simulink library "AEMS_Standard_Library"  (R2016b)
settings: Solver=ode45  StartTime=0.0  StopTime=10.0  RelTol=1e-3
undefined symbols (not defined in the file or in its folder): BkPY, carto, Cbx_extegr, Cbx_lpegrsys, Cbx_portegr, Cnx_bnk_nr_conf, Cnx_cyl_nr_conf, ConfigManagement, configuration_management, Cxx_dcm_io_tmr_end_xxxx, Cxx_dcm_rt_tmr_end, Cxx_DID_xxxx_IO_max, Cxx_DID_xxxx_IO_min, Cxx_egrhsofs, Cxx_vmaniegi, DEM_DEBOUNCE_FREEZE, DEM_DTR_CTL_INVISIBLE, DEM_DTR_CTL_NORMAL, Dem_DtrId2_XXX, Dem_DtrId3_XXX, Dem_DtrId4_XXX, Dem_DtrId5_XXX, Dem_DtrId6_XXX, Dem_DtrId7_XXX, Dem_DtrId8_XXX, Dem_DtrId9_XXX, Dem_DtrId_XXX, Dem_EnableConditionId2_XXX, Dem_EnableConditionId3_XXX, Dem_EnableConditionId4_XXX, Dem_EnableConditionId5_XXX, Dem_EnableConditionId6_XXX, Dem_EnableConditionId7_XXX, Dem_EnableConditionId8_XXX, Dem_EnableConditionId_XXX, Dem_EventId, Dem_EventId2_XXX, Dem_EventId3_XXX, Dem_EventId4_XXX, Dem_EventId5_XXX, Dem_EventId6_XXX, Dem_EventId7_XXX, Dem_EventId8_XXX, Dem_EventId9_XXX, Dem_EventId_Device_Faulttype, Dem_EventId_XXX, DEM_IUMPR_GENERAL_DENOMINATOR, DEM_OPCYC_IGNITION, Dem_RatioId2_XXX, Dem_RatioId3_XXX, Dem_RatioId4_XXX, Dem_RatioId5_XXX, Dem_RatioId6_XXX, Dem_RatioId7_XXX, Dem_RatioId8_XXX, Dem_RatioId_XXX, Dem_StorageConditionId2_XXX, Dem_StorageConditionId3_XXX, Dem_StorageConditionId4_XXX, Dem_StorageConditionId5_XXX ... (+65)
libraries: AEMS_Standard_Library x477, simulink x2
(part 10 of 39)

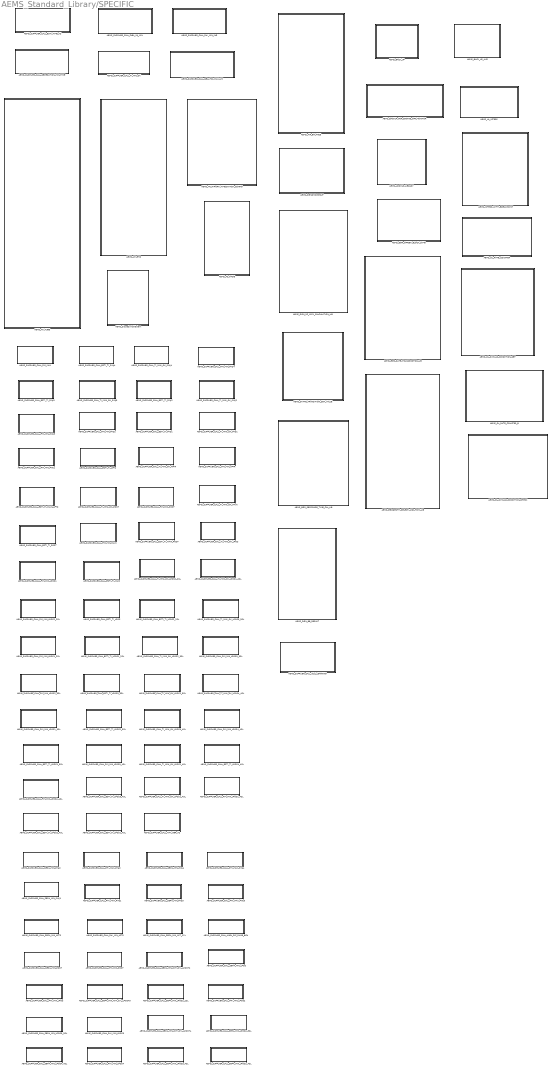
== system AEMS_Standard_Library/SPECIFIC ==
  AEMS_AIR_BALANCE : Subsystem  Tag=[LIB]  Description=User library of air balance calculation  mask(AEMS_AIR_BALANCE){Cnx_cyl_nr_conf=Cnx_cyl_nr_conf, Cbx_portegr=Cbx_portegr, Cbx_extegr=Cbx_extegr, Cxx_vmaniegi=Cxx_vmaniegi, Cbx_lpegrsys=Cbx_lpegrsys}
      mask prompts: Cnx_cyl_nr_conf "iCYLNDER"; Cbx_portegr "mfPORTEGR"; Cbx_extegr "mfEXTEGR"; Cxx_vmaniegi "mVMANIEGI"; Cbx_lpegrsys "mfLPEGRSYS"
      mask help:
      | Air Balance Block.
      | Use only at 2ms.
      settings: AttributesFormatString=%<MaskType>
      mask Help:
      | eval('path_lib=fileparts(which(''AEMS_Standard_Library''));');
      | doc_path = [path_lib '\help\AEMS_AIR_BALANCE.pdf'];
      | eval('open(doc_path)')
      mask Display: disp('AEMS_AIR_BALANCE')
  AEMS_AS_PADE : Subsystem  Tag=[LIB]  Description=|  TreatAsAtomicUnit=on  RTWFcnName=RSA_AS_Pade  mask(AEMS_AS_PADE){Cxb_lb_dly_t_para=Cxb_lb_dly_t_para, Cxp_lb_b0_1=Cxp_lb_b0_1, Cxp_lb_b1_1=Cxp_lb_b1_1, Cxp_lb_a1_1=Cxp_lb_a1_1, Cxp_lb_a2_1=Cxp_lb_a2_1, Cxp_lb_b0_2=Cxp_lb_b0_2, Cxp_lb_b1_2=Cxp_lb_b1_2, Cxp_lb_a1_2=Cxp_lb_a1_2, Cxp_lb_a2_2=Cxp_lb_a2_2, Cxp_lb_b0_3=Cxp_lb_b0_3, Cxp_lb_b1_3=Cxp_lb_b1_3, Cxp_lb_a1_3=Cxp_lb_a1_3, Cxp_lb_a2_3=Cxp_lb_a2_3}
      | This bloc describes a 6th-order Pade approximation of time delays.  It can be used to model dead times or transport delays in many processes.
      |                                                                                                                                              
      |  Inputs:                                                                                                                                     
      | Vbx_dly_ena:	 Boolean that enables the Pade delay model                                                                                      
      | Vbx_dly_init_ena:Boolean that initiates the Pade delay model                                                                                 
      | Vxx_dly_t:	delay time to be applied on the input signal (s)                                                                                  
      | Vxx_ftc_frst_order:	constant time of the upstream first order filter of Pade approximation  (s)                                              
      | Vxx_in:	 input signal to be delayed (kg/h)                                                                                                   
      |                                                                                                                                              
      | Outputs:                                                                                                                                     
      | Vxx_in_dly:            the approximation of delay time on the filtered input signal (kg/h)                                                   
      | Vxx_in_fil:              the input signal filtered by the first order filter (kg/h)
      mask help:
      | This block describes a 6th-order Pade approximation of time delays.  It can be used to model dead times or transport delays in many processes.
      |
      | Inputs:
      | Vbx_dly_init_ena:                Boolean that initiates the Pade delay model
      | Vxx_dly_t:                       Delay time to be applied on the input signal (s)
      | Vxx_ftc_frst_order:              Constant time of the upstream first order filter of Pade approximation  (s)
      | Vxx_in:                          Input signal to be delayed (kg/h)or (mg/strk)
      | Timestep:                        Time input that initiates the Pade delay model
      |
      | Outputs:
      | Vxx_in_dly:                      The approximation of delay time on the filtered input signal (kg/h) or (mg/strk)
      | Vxx_in_fil:                      The input signal filtered by the first order filter (kg/h) or (mg/strk)
      settings: AttributesFormatString=%<MaskType>\nCxb_lb_dly_t_para = %<Cxb_lb_dly_t_para>\nCxp_lb_b0_1 = %<Cxp_lb_b0_1>\nCxp_lb_b1_1 = %<Cxp_lb_b1_1>\nCxp_lb_a1_1 = %<Cxp_lb_a1_1>\nCxp_lb_a2_1 = %<Cxp_lb_a2_1>\nCxp_lb_b0_2 = %<Cxp_lb_b0_2>\nCxp_lb_b1_2 = %<Cxp_lb_b1_2>\nCxp_lb_a1_2 = %<Cxp_lb_a1_2>\nCxp_lb_a2_2 = %<Cxp_lb_a2_2>\nCxp_lb_b0_3 = %<Cxp_lb_b0_3>\nCxp_lb_b1_3 = %<Cxp_lb_b1_3>\nCxp_lb_a1_3 = %<Cxp_lb_a1_3>\nCxp_lb_a2_3 = %<Cxp_lb_a2_3>  RTWFcnNameOpts=User specified
      mask Help:
      | eval('path_lib=fileparts(which(''AEMS_Standard_Library''));');
      | mskblk=get_param(gcbh,'MaskType');
      | doc_path = [path_lib '\Help\',mskblk,'.pdf'];
      | eval('open(doc_path)');
      mask Display: disp('AEMS_AS_PADE\n\n')
  AEMS_AT_EHR : Subsystem  Tag=[LIB]  RTWFcnName=RSA_AT_ehr  mask(AEMS_AT_EHR){Den_Tol=1.1920929e-07}
      mask prompts: Den_Tol "Denominator Tolerance"
      mask help:
      | Library : thermal model
      | This function computes an energetic balance of the considered system. It estimates the brick temperature, the energy incoming, the energy leaving, the loss by external convection and the energy
      | created in the system.
      |
      | Version : 01.00
      settings: AttributesFormatString=%<MaskType>\nDenominator Tolerance=%<Den_Tol>  RTWFcnNameOpts=User specified
      mask Help:
      | eval('path_lib=fileparts(which(''AEMS_Standard_Library''));');
      | mskblk=get_param(gcbh,'MaskType');
      | doc_path = [path_lib '\Help\',mskblk,'.pdf'];
      | eval('open(doc_path)');
      mask Display: disp('AEMS_AT_EHR')
  AEMS_AT_TUBE : Subsystem  Tag=[LIB]  Description=|  RTWFcnName=RSA_AT_tube  mask(AEMS_AT_TUBE){Den_Tol=1.1920929e-07}
      | This block determines the exhaust gas downstream temperature, the temperature of the tube material,
      | the thermal power lost by the tube material and the thermal power lost by the gas inside the tube.
      mask prompts: Den_Tol "Denominator Tolerance"
      mask help:
      | This block determines the exhaust gas downstream temperature, the temperature of the tube material,
      | the thermal power lost by the tube material and the thermal power lost by the gas inside the tube.
      |
      | Version :01.00
      settings: AttributesFormatString=%<MaskType>\nDenominator Tolerance = %<Den_Tol>  RTWFcnNameOpts=User specified
      mask Help:
      | eval('path_lib=fileparts(which(''AEMS_Standard_Library''));');
      | mskblk=get_param(gcbh,'MaskType');
      | doc_path = [path_lib '\Help\',mskblk,'.pdf'];
      | eval('open(doc_path)');
      mask Display: disp('AEMS_AT_TUBE')
  AEMS_BACKUP_FOR_ENGINE_OFF_MONITOR : Subsystem  Tag=[LIB]  mask(AEMS_BACKUP_FOR_ENGINE_OFF_MONITOR){}
      mask help: This block is for Monitoring the Engine OFF condition.
      settings: AttributesFormatString=%<MaskType>
      mask Help:
      | eval('path_lib=fileparts(which(''AEMS_Standard_Library''));');
      | doc_path = [path_lib '\help\AEMS_BACKUP_FOR_ENGINE_OFF_MONITOR.pdf'];
      | eval('open(doc_path)')
      mask Display: disp('AEMS_BACKUP_FOR_ENGINE_OFF_MONITOR')
  AEMS_BACK_UP : Subsystem  Tag=[LIB]  mask(AEMS_BACK_UP){max_parameter=max, min_parameter=min}
      mask prompts: max_parameter "max"; min_parameter "min"
      mask init:
      | name=get_param(gcb,'MaskValueString');
      | name=sprintf(strrep(name,'|','\n'));
      | name=strread(name,'%s','delimiter',',');
      settings: AttributesFormatString=%<MaskType>\nmax = %<max_parameter>\nmin = %<min_parameter>
      mask Help:
      | eval('path_lib=fileparts(which(''AEMS_Standard_Library''));');
      | doc_path = [path_lib '\help\AEMS_BACK_UP.pdf'];
      | eval('open(doc_path)')
      mask Display: disp('AEMS_BACK_UP')
  AEMS_BACK_UP_AVE : Subsystem  Tag=[LIB]  mask(AEMS_BACK_UP_AVE){max_parameter=max, min_parameter=min}
      mask prompts: max_parameter "max"; min_parameter "min"
      mask init:
      | name=get_param(gcb,'MaskValueString');
      | name=sprintf(strrep(name,'|','\n'));
      | name=strread(name,'%s','delimiter',',');
      settings: AttributesFormatString=%<MaskType>\nmax = %<max_parameter>\nmin = %<min_parameter>
      mask Help:
      | eval('path_lib=fileparts(which(''AEMS_Standard_Library''));');
      | doc_path = [path_lib '\help\AEMS_BACK_UP_AVE.pdf'];
      | eval('open(doc_path)')
      mask Display: disp('AEMS_BACK_UP_AVE')
  AEMS_DGNDMDPGCUT : Subsystem  Tag=[LIB]  mask(AEMS_DGNDMDPGCUT){}
      settings: AttributesFormatString=%<MaskType>
      mask Help:
      | eval('path_lib=fileparts(which(''AEMS_Standard_Library''));');
      | doc_path = [path_lib '\help\AEMS_DGNDMDPGCUT.pdf'];
      | eval('open(doc_path)')
      mask Display: disp('AEMS_DGNDMDPGCUT')
  AEMS_DGN_BB_RESULT : Subsystem  Tag=[LIB]  mask(AEMS_DGN_BB_RESULT){}
      settings: AttributesFormatString=%<MaskType>
      mask Help:
      | eval('path_lib=fileparts(which(''AEMS_Standard_Library''));');
      | doc_path = [path_lib '\help\AEMS_DGN_BB_RESULT.pdf'];
      | eval('open(doc_path)')
      mask Display: disp('AEMS_DGN_BB_RESULT')
  AEMS_DGN_MF_MISX_CALCULATION_LIB : Subsystem  Tag=[LIB]  mask(AEMS_DGN_MF_MISX_CALCULATION_LIB){}
      settings: AttributesFormatString=%<MaskType>
      mask Help:
      | eval('path_lib=fileparts(which(''AEMS_Standard_Library''));');
      | doc_path = [path_lib '\help\AEMS_DGN_MF_MISX_CALCULATION_LIB.pdf'];
      | eval('open(doc_path)')
      mask Display: disp('AEMS_DGN_MF_MISX_CALCULATION_LIB')
  AEMS_EGRQESTH_SELECT_AND_TRIM_LIB : Subsystem  Tag=[LIB]  mask(AEMS_EGRQESTH_SELECT_AND_TRIM_LIB){}
      settings: AttributesFormatString=%<MaskType>
      mask Help:
      | eval('path_lib=fileparts(which(''AEMS_Standard_Library''));');
      | doc_path = [path_lib '\help\AEMS_EGRQESTH_SELECT_AND_TRIM_LIB.pdf'];
      | eval('open(doc_path)')
      mask Display: disp('AEMS_EGRQESTH_SELECT_AND_TRIM_LIB')
  AEMS_EGR_OFFSET_BLOCK_DIM8 : Subsystem  Tag=[LIB]  mask(AEMS_EGR_OFFSET_BLOCK_DIM8){Cxx_egrhsofs=0}
      mask prompts: Cxx_egrhsofs "mEGRHSOFS"
      settings: AttributesFormatString=%<MaskType>
      mask Help:
      | eval('path_lib=fileparts(which(''AEMS_Standard_Library''));');
      | doc_path = [path_lib '\help\AEMS_EGR_OFFSET_BLOCK_DIM8.pdf'];
      | eval('open(doc_path)')
      mask Display: disp('AEMS_EGR_OFFSET_BLOCK_DIM8')
  AEMS_EGR_RATE_TRANSPORTOR_LIB : Subsystem  Tag=[LIB]  Description=This USER LIBRARY calculates EGR rate delay of each part.  mask(AEMS_EGR_RATE_TRANSPORTOR_LIB){}
      mask help: This USER LIBRARY calculates EGR rate delay of each part.
      settings: AttributesFormatString=%<MaskType>
      mask Help:
      | eval('path_lib=fileparts(which(''AEMS_Standard_Library''));');
      | doc_path = [path_lib '\help\AEMS_EGR_RATE_TRANSPORTOR_LIB.pdf'];
      | eval('open(doc_path)')
      mask Display: disp('AEMS_EGR_RATE_TRANSPORTOR_LIB')
  AEMS_EGR_RESPONSE_TIME_CAL_LIB : Subsystem  Tag=[LIB]  mask(AEMS_EGR_RESPONSE_TIME_CAL_LIB){}
      settings: AttributesFormatString=%<MaskType>
      mask Help:
      | eval('path_lib=fileparts(which(''AEMS_Standard_Library''));');
      | doc_path = [path_lib '\help\AEMS_EGR_RESPONSE_TIME_CAL_LIB.pdf'];
      | eval('open(doc_path)')
      mask Display: disp('AEMS_EGR_RESPONSE_TIME_CAL_LIB')
  AEMS_INTERP_WITH_BREAKPOINT : Subsystem  Tag=[LIB]  mask(AEMS_INTERP_WITH_BREAKPOINT){}
      settings: AttributesFormatString=%<MaskType>
      mask Help:
      | eval('path_lib=fileparts(which(''AEMS_Standard_Library''));');
      | doc_path = [path_lib '\help\AEMS_INTERP_WITH_BREAKPOINT.pdf'];
      | eval('open(doc_path)')
      mask Display: disp('AEMS_INTERP_WITH_BREAKPOINT')
  AEMS_LOOKUP_LIBRARY : Subsystem  Tag=[LIB]  mask(AEMS_LOOKUP_LIBRARY){}
      settings: AttributesFormatString=%<MaskType>
      mask Help:
      | eval('path_lib=fileparts(which(''AEMS_Standard_Library''));');
      | doc_path = [path_lib '\help\AEMS_LOOKUP_LIBRARY.pdf'];
      | eval('open(doc_path)')
      mask Display: disp('AEMS_LOOKUP_LIBRARY')
  AEMS_MULTIPORT_TIMESWITCH_CONFIG : Subsystem  Tag=[LIB]  mask(AEMS_MULTIPORT_TIMESWITCH_CONFIG){LimitDimInputs=8}
      mask prompts: LimitDimInputs "Limit of Dimension of Inputs"
      mask help:
      | This switch allows to switch among inputs regrouped in a vector using Selector. It provides a smooth transition between the previously selected input and the currently selected input over a duration.
      | It should be noted that during the transition, the current value of both inputs is taken into account and not just values at the moment of switching.
      |
      | As a result, discontinuities can arise if a new input is seleted before the previous transition has ended.
      |
      | [INPUTS]
      | Duration: Transition duration
      | Select_Input: Select an input in the vector Inputs
      | Inputs: Regrouped inputs
      | dT: Sample time
      |
      | [OUTPUTS]
      | Output: Smooth value from previous and current selected inputs
      | Slop_on: indicate that there is a switch
      |
      | [PARAMETERS]
      | LimitNumberInputs: Limit number of input signals regrouped in Inputs
      settings: AttributesFormatString=|
      | %<MaskType>
      | Limit Dimension of Inputs : %<LimitDimInputs>
      mask Help:
      | eval('path_lib=fileparts(which(''lib_dcmap_sdt''));');
      | doc_path = [path_lib '\help\AEMS_MULTIPORT_TIMESWITCH_CONFIG.pdf'];
      | eval('open(doc_path)')
      mask Display: disp('AEMS_MULTIPORT_TIMESWITCH_CONFIG')
  AEMS_OL_RATE_COUNTER : Subsystem  Tag=[LIB]  mask(AEMS_OL_RATE_COUNTER){}
      settings: AttributesFormatString=%<MaskType>
      mask Help:
      | eval('path_lib=fileparts(which(''AEMS_Standard_Library''));');
      | doc_path = [path_lib '\help\AEMS_OL_RATE_COUNTER.pdf'];
      | eval('open(doc_path)')
      mask Display: disp('AEMS_OL_RATE_COUNTER')
  AEMS_OL_RATE_COUNTER_B : Subsystem  Tag=[LIB]  mask(AEMS_OL_RATE_COUNTER_B){}
      settings: AttributesFormatString=%<MaskType>
      mask Help:
      | eval('path_lib=fileparts(which(''AEMS_Standard_Library''));');
      | doc_path = [path_lib '\help\AEMS_OL_RATE_COUNTER_B.pdf'];
      | eval('open(doc_path)')
      mask Display: disp('AEMS_OL_RATE_COUNTER_B')
  AEMS_OL_SIMILAR_CONDITION_CHECK : Subsystem  Tag=[LIB]  mask(AEMS_OL_SIMILAR_CONDITION_CHECK){}
      settings: AttributesFormatString=%<MaskType>
      mask Help:
      | eval('path_lib=fileparts(which(''AEMS_Standard_Library''));');
      | doc_path = [path_lib '\help\AEMS_OL_SIMILAR_CONDITION_CHECK.pdf'];
      | eval('open(doc_path)')
      mask Display: disp('AEMS_OL_SIMILAR_CONDITION_CHECK')
  AEMS_OL_SIMILAR_CONDITION_SET : Subsystem  Tag=[LIB]  mask(AEMS_OL_SIMILAR_CONDITION_SET){}
      settings: AttributesFormatString=%<MaskType>
      mask Help:
      | eval('path_lib=fileparts(which(''AEMS_Standard_Library''));');
      | doc_path = [path_lib '\help\AEMS_OL_SIMILAR_CONDITION_SET.pdf'];
      | eval('open(doc_path)')
      mask Display: disp('AEMS_OL_SIMILAR_CONDITION_SET')
  AEMS_STATE_TRANSITION_SET_VALUE : Subsystem  Tag=[LIB]  mask(AEMS_STATE_TRANSITION_SET_VALUE){}
      settings: AttributesFormatString=%<MaskType>
      mask Help:
      | eval('path_lib=fileparts(which(''AEMS_Standard_Library''));');
      | doc_path = [path_lib '\help\AEMS_STATE_TRANSITION_SET_VALUE.pdf'];
      | eval('open(doc_path)')
      mask Display: disp('AEMS_STATE_TRANSITION_SET_VALUE')
  AEMS_SUPPLIER_CALL_ANGL_DIF_SAME_BCH : Subsystem  Tag=[LIB]  TreatAsAtomicUnit=on  RTWFcnName=SUPPLIER_CALL_Angl_dif_same_bch  mask(AEMS_SUPPLIER_CALL_ANGL_DIF_SAME_BCH){}
      mask help: Angle without injection command between 2 cylinder ordered by the same bench.
      mask init:
      | Thisblk = gcb;
      | model_type_pos = strsplit(Thisblk,'/');%to split all the layer paths in order to get the runnable path
      | runnable_path = [bdroot '/' model_type_pos{2}];%to get the runnable or AIPCALL path
      | trg_port_name = get_param(find_system(runnable_path,'BlockType','TriggerPort'),'Name');%to get the function call trigger name
      | TaskRate = '';%the raster suffix is stored in the parameter 
      | 
      | if ~isempty(trg_port_name)
      |     trg_port_name_spltd = strsplit(trg_port_name{1},'_');%splitting is done in order to get the raster and its type(Sched or Event)
      |     
      |     % checking for rasters of type Sched or Event especially occuring in
      |     % runnables
      |     if ~isempty(regexp(trg_port_name_spltd{1},'^Sched|^Event','once')) 
      |         TaskRate = ['_' regexprep(trg_port_name_spltd{1},'Sched|Event','','once')];
      |         
      |     %checking if the raster is dcmcb and this is applicable only for
      |     %APICALL
      |     elseif ~isempty(regexp([trg_port_name_spltd{1} '_' trg_port_name_spltd{2} '_' ],'^DataServices_DCM_|^RoutineServices_DCM_','once'))||...
      |             ~isempty(regexp(trg_port_name_spltd{1},'^Dcm$','once'))
      |         TaskRate = '_dcmcb';
      |         
      |     %checking if this block is used under the function call trigger
      |     %starting with "Com" and then giving an error message
      |     %this is applicable only for APICALL
      |     elseif ~isempty(regexp(trg_port_name_spltd{1},'^Com$','once'))
      |         msg = sprintf(['\n','The Supplier call block "' Thisblk '" should not be present within APICALLs having function call trigger as "Com"']);
      |         errordlg(msg);
      |         return;
      |     end
      | end
      | 
      | DataName = ['Supplier_call_angl_dif_nxt_cyl' TaskRate];%the variable name that should be given to DataStoreRead block 
      | set_param([Thisblk '/DataStoreRead'],'DataStoreName',DataName);%Setting the DataStoreName of DataStoreRead block
      | 
      | %other settings done to this variable name
      | structVxx=Simulink.Signal;
      | structVxx.Dimensions=1;
      | structVxx.DimensionsMode='Fixed';
      | structVxx.DataType='single';
      | structVxx.Complexity='real';
      | structVxx.SamplingMode='Sample based';
      | structVxx.SampleTime=-1;
      | assignin('base',DataName,structVxx);
      settings: AttributesFormatString=%<MaskType>  RTWSystemCode=Nonreusable function  RTWFcnNameOpts=User specified
      mask Help:
      | eval('path_lib=fileparts(which(''AEMS_Standard_Library''));');
      | mskblk=get_param(gcbh,'MaskType');
      | doc_path = [path_lib '\Help\',mskblk,'.pdf'];
      | eval('open(doc_path)');
  AEMS_SUPPLIER_CALL_ESTI_TIME_INJ : Subsystem  Tag=[LIB]  TreatAsAtomicUnit=on  RTWFcnName=SUPPLIER_CALL_Esti_ti_main_post3  mask(AEMS_SUPPLIER_CALL_ESTI_TIME_INJ){Outportname=Vxx_fms_esti_ti_wish_main_post2, Suppliercallname=SUPPLIER_CALL_Esti_ti_main_post2, Splitnum=2}
      mask prompts: Outportname "Outport Name"; Suppliercallname "Supplier call Name"; Splitnum "Split"
      mask help:
      | Estimation of time of injection, depending on rail pressure, on fuel quantity and of fuel density.
      |
      | Each block will be translated into code C by this way:
      | Output=Supplier call API Name(In,Splitnum);
      | Example for Supplier_Call_Esti_ti_main_post3, corresponding output variable is Vxx_fms_esti_ti_wish_main_post3
      | Vxx_fms_esti_ti_wish_main_post3= Supplier_Call_Esti_ti_main_post3(In,3);
      mask init:
      | ThisBlk = gcb;
      | OutPorts            =   {'Vxx_fms_esti_ti_post1','Vxx_fms_esti_ti_post1_2sl','Vxx_fms_esti_ti_post1_3sl','Vxx_fms_esti_ti_post2_2sl','Vxx_fms_esti_ti_post2_3sl',...
      |                     'Vxx_fms_esti_ti_post3_3sl','Vxx_fms_esti_ti_wish_main_post1','Vxx_fms_esti_ti_wish_main_post2','Vxx_fms_esti_ti_wish_main_post3'};
      | 
      | Supplier_Calls      =   {'SUPPLIER_CALL_Esti_ti_post1','SUPPLIER_CALL_Esti_ti_post1','SUPPLIER_CALL_Esti_ti_post1','SUPPLIER_CALL_Esti_ti_post2','SUPPLIER_CALL_Esti_ti_post2',...
      |                           'SUPPLIER_CALL_Esti_ti_post3','SUPPLIER_CALL_Esti_ti_main_post1','SUPPLIER_CALL_Esti_ti_main_post2','SUPPLIER_CALL_Esti_ti_main_post3'};
      | 
      | Data_Names         =   {'Supplier_Call_Esti_ti_post1','Supplier_Call_Esti_ti_post1','Supplier_Call_Esti_ti_post1','Supplier_Call_Esti_ti_post2','Supplier_Call_Esti_ti_post2',...
      |                           'Supplier_Call_Esti_ti_post3','Supplier_Call_Esti_ti_main_post1','Supplier_Call_Esti_ti_main_post2','Supplier_Call_Esti_ti_main_post3'};                      
      |                       
      |                       
      | Splits              =   {'1','2','3','2','3','3','1','2','3'};
      | 
      | model_type_pos = strsplit(ThisBlk,'/');
      | runnable_path = [bdroot '/' model_type_pos{2}];%to get the runnable or AIPCALL path
      | trg_port_name = get_param(find_system(runnable_path,'BlockType','TriggerPort'),'Name');%to get the function call trigger name
      | TaskRate = '';
      | if ~isempty(trg_port_name)
      |     trg_port_name_spltd = strsplit(trg_port_name{1},'_');
      |     if ~isempty(regexp(trg_port_name_spltd{1},'^Sched|^Event','once'))
      |         TaskRate = ['_' regexprep(trg_port_name_spltd{1},'Sched|Event','','once')];
      |     elseif ~isempty(regexp([trg_port_name_spltd{1} '_' trg_port_name_spltd{2} '_' ],'^DataServices_DCM_|^RoutineServices_DCM_','once'))||...
      |             ~isempty(regexp(trg_port_name_spltd{1},'^Dcm$','once'))
      |         TaskRate = '_dcmcb';
      |     elseif ~isempty(regexp(trg_port_name_spltd{1},'^Com$','once'))
      |         msg = sprintf(['\n','The Supplier call block "' Thisblk '" should not be present within APICALLs having function call trigger as "Com"']);
      |         errordlg(msg);
      |         return;
      |     end
      | end
      | 
      | Idx_Of_Outportname = find(ismember(OutPorts,Outportname));
      | DataName = [Data_Names{Idx_Of_Outportname} TaskRate];
      | 
      | %set the  suppliername according to the Outport name.
      | set_param(ThisBlk,'Suppliercallname',Supplier_Calls{Idx_Of_Outportname});
      | set_param(ThisBlk,'Splitnum',Splits{Idx_Of_Outportname});
      | 
      | %Get the paths of the blks under this lib block.
      | Const_Blk = [ThisBlk,'/Splitnum'];%%path of "const block" inside this lib blk.
      | DSR_Blk   = [ThisBlk,'/Data_Store_Read'];%path of "Data store read block" inside this lib blk.
      | Outport_Blk = find_system(ThisBlk,'LookUnderMasks','all','FollowLinks','on','BlockType','Outport');
      | Outport_Blk = Outport_Blk{1};%I know this is d only outport blk.
      | 
      | %set the attributes of the blks under this lib block, based on teh Outportname chosen by d user.
      | set_param(Outport_Blk,'Name',Outportname);
      | set_param(DSR_Blk,'DataStoreName',DataName);
      | set_param(Const_Blk,'Value',Splits{Idx_Of_Outportname});
      | 
      | %To create a singal object in d base workspace.
      | EvalStr = ['exist(''',DataName,''',''var'')'];
      | structVxx=Simulink.Signal;
      | structVxx.Dimensions=1;
      | structVxx.DimensionsMode='Fixed';
      | structVxx.DataType='single';
      | structVxx.Complexity='real';
      | structVxx.SamplingMode='Sample based';
      | structVxx.SampleTime=-1;
      | isDefined= evalin('base',EvalStr);%This line checks whether the DataName exist in the base workspace.
      | if (isDefined==0)
      |     assignin('base',DataName,structVxx);
      | end
      settings: RTWSystemCode=Inline  RTWFcnNameOpts=User specified
      settings: AttributesFormatString=|
      | %<MaskType>
      | Supplier Call Name = %<Suppliercallname>
      | Outport Name = %<Outportname>
      | Split Number = %<Splitnum>
      mask Help:
      | eval('path_lib=fileparts(which(''AEMS_Standard_Library''));');
      | mskblk=get_param(gcbh,'MaskType');
      | doc_path = [path_lib '\Help\',mskblk,'.pdf'];
      | eval('open(doc_path)');
      mask TypeOptions Outportname: Vxx_fms_esti_ti_post1 | Vxx_fms_esti_ti_post1_2sl | Vxx_fms_esti_ti_post1_3sl | Vxx_fms_esti_ti_post2_2sl | Vxx_fms_esti_ti_post2_3sl | Vxx_fms_esti_ti_post3_3sl | Vxx_fms_esti_ti_wish_main_post1 | Vxx_fms_esti_ti_wish_main_post2 | Vxx_fms_esti_ti_wish_main_post3
      mask Callback Outportname:
      | OutPorts            =   {'Vxx_fms_esti_ti_post1','Vxx_fms_esti_ti_post1_2sl','Vxx_fms_esti_ti_post1_3sl','Vxx_fms_esti_ti_post2_2sl','Vxx_fms_esti_ti_post2_3sl',...
      |                     'Vxx_fms_esti_ti_post3_3sl','Vxx_fms_esti_ti_wish_main_post1','Vxx_fms_esti_ti_wish_main_post2','Vxx_fms_esti_ti_wish_main_post3'};
      | 
      | Supplier_Calls      =   {'SUPPLIER_CALL_Esti_ti_post1','SUPPLIER_CALL_Esti_ti_post1','SUPPLIER_CALL_Esti_ti_post1','SUPPLIER_CALL_Esti_ti_post2','SUPPLIER_CALL_Esti_ti_post2',...
      |                           'SUPPLIER_CALL_Esti_ti_post3','SUPPLIER_CALL_Esti_ti_main_post1','SUPPLIER_CALL_Esti_ti_main_post2','SUPPLIER_CALL_Esti_ti_main_post3'};
      | 
      | Splits              =   {'1','2','3','2','3','3','1','2','3'};
      | 
      | Outportname = get_param(gcb,'Outportname');
      | 
      | Idx_Of_Outportname = find(ismember(OutPorts,Outportname));
      | %set the  suppliername according to the Outport name.
      | set_param(gcb,'Suppliercallname',Supplier_Calls{Idx_Of_Outportname});
      | set_param(gcb,'Splitnum',Splits{Idx_Of_Outportname});
      | cellfun(@clear,{'Idx_Of_Outportname','Outportname','OutPorts','Splits','Supplier_Calls'});
  AEMS_SUPPLIER_CALL_ESTI_TI_AFTR : Subsystem  Tag=[LIB]  TreatAsAtomicUnit=on  RTWFcnName=SUPPLIER_CALL_Esti_ti_aftr  mask(AEMS_SUPPLIER_CALL_ESTI_TI_AFTR){}
      mask help:
      | Estimation of time of injection, depending on rail pressure, on fuel quantity and of fuel density
      |
      | This block is to call Supplier call API.
      mask init:
      | Thisblk = gcb;
      | model_type_pos = strsplit(Thisblk,'/');%to split all the layer paths in order to get the runnable path
      | runnable_path = [bdroot '/' model_type_pos{2}];%to get the runnable or AIPCALL path
      | trg_port_name = get_param(find_system(runnable_path,'BlockType','TriggerPort'),'Name');%to get the function call trigger name
      | TaskRate = '';%the raster suffix is stored in the parameter 
      | 
      | if ~isempty(trg_port_name)
      |     trg_port_name_spltd = strsplit(trg_port_name{1},'_');%splitting is done in order to get the raster and its type(Sched or Event)
      |     
      |     % checking for rasters of type Sched or Event especially occuring in
      |     % runnables
      |     if ~isempty(regexp(trg_port_name_spltd{1},'^Sched|^Event','once')) 
      |         TaskRate = ['_' regexprep(trg_port_name_spltd{1},'Sched|Event','','once')];
      |         
      |     %checking if the raster is dcmcb and this is applicable only for
      |     %APICALL
      |     elseif ~isempty(regexp([trg_port_name_spltd{1} '_' trg_port_name_spltd{2} '_' ],'^DataServices_DCM_|^RoutineServices_DCM_','once'))||...
      |             ~isempty(regexp(trg_port_name_spltd{1},'^Dcm$','once'))
      |         TaskRate = '_dcmcb';
      |         
      |     %checking if this block is used under the function call trigger
      |     %starting with "Com" and then giving an error message
      |     %this is applicable only for APICALL
      |     elseif ~isempty(regexp(trg_port_name_spltd{1},'^Com$','once'))
      |         msg = sprintf(['\n','The Supplier call block "' Thisblk '" should not be present within APICALLs having function call trigger as "Com"']);
      |         errordlg(msg);
      |         return;
      |     end
      | end
      | 
      | DataName = ['Supplier_call_esti_ti_aftr' TaskRate];%the variable name that should be given to DataStoreRead block 
      | set_param([Thisblk '/DataStoreRead'],'DataStoreName',DataName);%Setting the DataStoreName of DataStoreRead block
      | 
      | %other settings done to this variable name
      | structVxx=Simulink.Signal;
      | structVxx.Dimensions=1;
      | structVxx.DimensionsMode='Fixed';
      | structVxx.DataType='single';
      | structVxx.Complexity='real';
      | structVxx.SamplingMode='Sample based';
      | structVxx.SampleTime=-1;
      | assignin('base',DataName,structVxx);
      settings: AttributesFormatString=%<MaskType>  RTWSystemCode=Nonreusable function  RTWFcnNameOpts=User specified
      mask Help:
      | eval('path_lib=fileparts(which(''AEMS_Standard_Library''));');
      | mskblk=get_param(gcbh,'MaskType');
      | doc_path = [path_lib '\Help\',mskblk,'.pdf'];
      | eval('open(doc_path)');
  AEMS_SUPPLIER_CALL_ESTI_TI_LPOS : Subsystem  Tag=[LIB]  TreatAsAtomicUnit=on  RTWFcnName=SUPPLIER_CALL_Esti_ti_lpos  mask(AEMS_SUPPLIER_CALL_ESTI_TI_LPOS){}
      mask help:
      | Estimation of time of injection, depending on rail pressure, on fuel quantity and of fuel density
      |
      | This block is to call Supplier call API.
      mask init:
      | Thisblk = gcb;
      | model_type_pos = strsplit(Thisblk,'/');%to split all the layer paths in order to get the runnable path
      | runnable_path = [bdroot '/' model_type_pos{2}];%to get the runnable or AIPCALL path
      | trg_port_name = get_param(find_system(runnable_path,'BlockType','TriggerPort'),'Name');%to get the function call trigger name
      | TaskRate = '';%the raster suffix is stored in the parameter 
      | 
      | if ~isempty(trg_port_name)
      |     trg_port_name_spltd = strsplit(trg_port_name{1},'_');%splitting is done in order to get the raster and its type(Sched or Event)
      |     
      |     % checking for rasters of type Sched or Event especially occuring in
      |     % runnables
      |     if ~isempty(regexp(trg_port_name_spltd{1},'^Sched|^Event','once')) 
      |         TaskRate = ['_' regexprep(trg_port_name_spltd{1},'Sched|Event','','once')];
      |         
      |     %checking if the raster is dcmcb and this is applicable only for
      |     %APICALL
      |     elseif ~isempty(regexp([trg_port_name_spltd{1} '_' trg_port_name_spltd{2} '_' ],'^DataServices_DCM_|^RoutineServices_DCM_','once'))||...
      |             ~isempty(regexp(trg_port_name_spltd{1},'^Dcm$','once'))
      |         TaskRate = '_dcmcb';
      |         
      |     %checking if this block is used under the function call trigger
      |     %starting with "Com" and then giving an error message
      |     %this is applicable only for APICALL
      |     elseif ~isempty(regexp(trg_port_name_spltd{1},'^Com$','once'))
      |         msg = sprintf(['\n','The Supplier call block "' Thisblk '" should not be present within APICALLs having function call trigger as "Com"']);
      |         errordlg(msg);
      |         return;
      |     end
      | end
      | 
      | DataName = ['Supplier_call_esti_ti_lpos' TaskRate];%the variable name that should be given to DataStoreRead block 
      | set_param([Thisblk '/DataStoreRead'],'DataStoreName',DataName);%Setting the DataStoreName of DataStoreRead block
      | 
      | %other settings done to this variable name
      | structVxx=Simulink.Signal;
      | structVxx.Dimensions=1;
      | structVxx.DimensionsMode='Fixed';
      | structVxx.DataType='single';
      | structVxx.Complexity='real';
      | structVxx.SamplingMode='Sample based';
      | structVxx.SampleTime=-1;
      | assignin('base',DataName,structVxx);
      settings: AttributesFormatString=%<MaskType>  RTWSystemCode=Nonreusable function  RTWFcnNameOpts=User specified
      mask Help:
      | eval('path_lib=fileparts(which(''AEMS_Standard_Library''));');
      | mskblk=get_param(gcbh,'MaskType');
      | doc_path = [path_lib '\Help\',mskblk,'.pdf'];
      | eval('open(doc_path)');
  AEMS_SUPPLIER_CALL_ESTI_TI_LPOS1_2SL : Subsystem  Tag=[LIB]  TreatAsAtomicUnit=on  RTWFcnName=SUPPLIER_CALL_Esti_ti_lpos1_2sl  mask(AEMS_SUPPLIER_CALL_ESTI_TI_LPOS1_2SL){}
      mask help:
      | Estimation of time of injection, depending on rail pressure, on fuel quantity and of fuel density
      |
      | This block is to call Supplier call API.
      mask init:
      | Thisblk = gcb;
      | model_type_pos = strsplit(Thisblk,'/');%to split all the layer paths in order to get the runnable path
      | runnable_path = [bdroot '/' model_type_pos{2}];%to get the runnable or AIPCALL path
      | trg_port_name = get_param(find_system(runnable_path,'BlockType','TriggerPort'),'Name');%to get the function call trigger name
      | TaskRate = '';%the raster suffix is stored in the parameter 
      | 
      | if ~isempty(trg_port_name)
      |     trg_port_name_spltd = strsplit(trg_port_name{1},'_');%splitting is done in order to get the raster and its type(Sched or Event)
      |     
      |     % checking for rasters of type Sched or Event especially occuring in
      |     % runnables
      |     if ~isempty(regexp(trg_port_name_spltd{1},'^Sched|^Event','once')) 
      |         TaskRate = ['_' regexprep(trg_port_name_spltd{1},'Sched|Event','','once')];
      |         
      |     %checking if the raster is dcmcb and this is applicable only for
      |     %APICALL
      |     elseif ~isempty(regexp([trg_port_name_spltd{1} '_' trg_port_name_spltd{2} '_' ],'^DataServices_DCM_|^RoutineServices_DCM_','once'))||...
      |             ~isempty(regexp(trg_port_name_spltd{1},'^Dcm$','once'))
      |         TaskRate = '_dcmcb';
      |         
      |     %checking if this block is used under the function call trigger
      |     %starting with "Com" and then giving an error message
      |     %this is applicable only for APICALL
      |     elseif ~isempty(regexp(trg_port_name_spltd{1},'^Com$','once'))
      |         msg = sprintf(['\n','The Supplier call block "' Thisblk '" should not be present within APICALLs having function call trigger as "Com"']);
      |         errordlg(msg);
      |         return;
      |     end
      | end
      | 
      | DataName = ['Supplier_call_esti_ti_lpos1_2sl' TaskRate];%the variable name that should be given to DataStoreRead block 
      | set_param([Thisblk '/DataStoreRead'],'DataStoreName',DataName);%Setting the DataStoreName of DataStoreRead block
      | 
      | %other settings done to this variable name
      | structVxx=Simulink.Signal;
      | structVxx.Dimensions=1;
      | structVxx.DimensionsMode='Fixed';
      | structVxx.DataType='single';
      | structVxx.Complexity='real';
      | structVxx.SamplingMode='Sample based';
      | structVxx.SampleTime=-1;
      | assignin('base',DataName,structVxx);
      settings: AttributesFormatString=%<MaskType>  RTWSystemCode=Nonreusable function  RTWFcnNameOpts=User specified
      mask Help:
      | eval('path_lib=fileparts(which(''AEMS_Standard_Library''));');
      | mskblk=get_param(gcbh,'MaskType');
      | doc_path = [path_lib '\Help\',mskblk,'.pdf'];
      | eval('open(doc_path)');
  AEMS_SUPPLIER_CALL_ESTI_TI_LPOS1_3SL : Subsystem  Tag=[LIB]  TreatAsAtomicUnit=on  RTWFcnName=SUPPLIER_CALL_Esti_ti_lpos1_3sl  mask(AEMS_SUPPLIER_CALL_ESTI_TI_LPOS1_3SL){}
      mask help:
      | Estimation of time of injection, depending on rail pressure, on fuel quantity and of fuel density
      |
      | This block is to call Supplier call API.
      mask init:
      | Thisblk = gcb;
      | model_type_pos = strsplit(Thisblk,'/');%to split all the layer paths in order to get the runnable path
      | runnable_path = [bdroot '/' model_type_pos{2}];%to get the runnable or AIPCALL path
      | trg_port_name = get_param(find_system(runnable_path,'BlockType','TriggerPort'),'Name');%to get the function call trigger name
      | TaskRate = '';%the raster suffix is stored in the parameter 
      | 
      | if ~isempty(trg_port_name)
      |     trg_port_name_spltd = strsplit(trg_port_name{1},'_');%splitting is done in order to get the raster and its type(Sched or Event)
      |     
      |     % checking for rasters of type Sched or Event especially occuring in
      |     % runnables
      |     if ~isempty(regexp(trg_port_name_spltd{1},'^Sched|^Event','once')) 
      |         TaskRate = ['_' regexprep(trg_port_name_spltd{1},'Sched|Event','','once')];
      |         
      |     %checking if the raster is dcmcb and this is applicable only for
      |     %APICALL
      |     elseif ~isempty(regexp([trg_port_name_spltd{1} '_' trg_port_name_spltd{2} '_' ],'^DataServices_DCM_|^RoutineServices_DCM_','once'))||...
      |             ~isempty(regexp(trg_port_name_spltd{1},'^Dcm$','once'))
      |         TaskRate = '_dcmcb';
      |         
      |     %checking if this block is used under the function call trigger
      |     %starting with "Com" and then giving an error message
      |     %this is applicable only for APICALL
      |     elseif ~isempty(regexp(trg_port_name_spltd{1},'^Com$','once'))
      |         msg = sprintf(['\n','The Supplier call block "' Thisblk '" should not be present within APICALLs having function call trigger as "Com"']);
      |         errordlg(msg);
      |         return;
      |     end
      | end
      | 
      | DataName = ['Supplier_call_esti_ti_lpos1_3sl' TaskRate];%the variable name that should be given to DataStoreRead block 
      | set_param([Thisblk '/DataStoreRead'],'DataStoreName',DataName);%Setting the DataStoreName of DataStoreRead block
      | 
      | %other settings done to this variable name
      | structVxx=Simulink.Signal;
      | structVxx.Dimensions=1;
      | structVxx.DimensionsMode='Fixed';
      | structVxx.DataType='single';
      | structVxx.Complexity='real';
      | structVxx.SamplingMode='Sample based';
      | structVxx.SampleTime=-1;
      | assignin('base',DataName,structVxx);
      settings: AttributesFormatString=%<MaskType>  RTWSystemCode=Nonreusable function  RTWFcnNameOpts=User specified
      mask Help:
      | eval('path_lib=fileparts(which(''AEMS_Standard_Library''));');
      | mskblk=get_param(gcbh,'MaskType');
      | doc_path = [path_lib '\Help\',mskblk,'.pdf'];
      | eval('open(doc_path)');
  AEMS_SUPPLIER_CALL_ESTI_TI_LPOS1_4SL : Subsystem  Tag=[LIB]  TreatAsAtomicUnit=on  RTWFcnName=SUPPLIER_CALL_Esti_ti_lpos1_4sl  mask(AEMS_SUPPLIER_CALL_ESTI_TI_LPOS1_4SL){}
      mask help:
      | Estimation of time of injection, depending on rail pressure, on fuel quantity and of fuel density
      |
      | This block is to call Supplier call API.
      mask init:
      | Thisblk = gcb;
      | model_type_pos = strsplit(Thisblk,'/');%to split all the layer paths in order to get the runnable path
      | runnable_path = [bdroot '/' model_type_pos{2}];%to get the runnable or AIPCALL path
      | trg_port_name = get_param(find_system(runnable_path,'BlockType','TriggerPort'),'Name');%to get the function call trigger name
      | TaskRate = '';%the raster suffix is stored in the parameter 
      | 
      | if ~isempty(trg_port_name)
      |     trg_port_name_spltd = strsplit(trg_port_name{1},'_');%splitting is done in order to get the raster and its type(Sched or Event)
      |     
      |     % checking for rasters of type Sched or Event especially occuring in
      |     % runnables
      |     if ~isempty(regexp(trg_port_name_spltd{1},'^Sched|^Event','once')) 
      |         TaskRate = ['_' regexprep(trg_port_name_spltd{1},'Sched|Event','','once')];
      |         
      |     %checking if the raster is dcmcb and this is applicable only for
      |     %APICALL
      |     elseif ~isempty(regexp([trg_port_name_spltd{1} '_' trg_port_name_spltd{2} '_' ],'^DataServices_DCM_|^RoutineServices_DCM_','once'))||...
      |             ~isempty(regexp(trg_port_name_spltd{1},'^Dcm$','once'))
      |         TaskRate = '_dcmcb';
      |         
      |     %checking if this block is used under the function call trigger
      |     %starting with "Com" and then giving an error message
      |     %this is applicable only for APICALL
      |     elseif ~isempty(regexp(trg_port_name_spltd{1},'^Com$','once'))
      |         msg = sprintf(['\n','The Supplier call block "' Thisblk '" should not be present within APICALLs having function call trigger as "Com"']);
      |         errordlg(msg);
      |         return;
      |     end
      | end
      | 
      | DataName = ['Supplier_call_esti_ti_lpos1_4sl' TaskRate];%the variable name that should be given to DataStoreRead block 
      | set_param([Thisblk '/DataStoreRead'],'DataStoreName',DataName);%Setting the DataStoreName of DataStoreRead block
      | 
      | %other settings done to this variable name
      | structVxx=Simulink.Signal;
      | structVxx.Dimensions=1;
      | structVxx.DimensionsMode='Fixed';
      | structVxx.DataType='single';
      | structVxx.Complexity='real';
      | structVxx.SamplingMode='Sample based';
      | structVxx.SampleTime=-1;
      | assignin('base',DataName,structVxx);
      settings: AttributesFormatString=%<MaskType>  RTWSystemCode=Nonreusable function  RTWFcnNameOpts=User specified
      mask Help:
      | eval('path_lib=fileparts(which(''AEMS_Standard_Library''));');
      | mskblk=get_param(gcbh,'MaskType');
      | doc_path = [path_lib '\Help\',mskblk,'.pdf'];
      | eval('open(doc_path)');
  AEMS_SUPPLIER_CALL_ESTI_TI_LPOS2_2SL : Subsystem  Tag=[LIB]  TreatAsAtomicUnit=on  RTWFcnName=SUPPLIER_CALL_Esti_ti_lpos2_2sl  mask(AEMS_SUPPLIER_CALL_ESTI_TI_LPOS2_2SL){}
      mask help:
      | Estimation of time of injection, depending on rail pressure, on fuel quantity and of fuel density
      |
      | This block is to call Supplier call API.
      mask init:
      | Thisblk = gcb;
      | model_type_pos = strsplit(Thisblk,'/');%to split all the layer paths in order to get the runnable path
      | runnable_path = [bdroot '/' model_type_pos{2}];%to get the runnable or AIPCALL path
      | trg_port_name = get_param(find_system(runnable_path,'BlockType','TriggerPort'),'Name');%to get the function call trigger name
      | TaskRate = '';%the raster suffix is stored in the parameter 
      | 
      | if ~isempty(trg_port_name)
      |     trg_port_name_spltd = strsplit(trg_port_name{1},'_');%splitting is done in order to get the raster and its type(Sched or Event)
      |     
      |     % checking for rasters of type Sched or Event especially occuring in
      |     % runnables
      |     if ~isempty(regexp(trg_port_name_spltd{1},'^Sched|^Event','once')) 
      |         TaskRate = ['_' regexprep(trg_port_name_spltd{1},'Sched|Event','','once')];
      |         
      |     %checking if the raster is dcmcb and this is applicable only for
      |     %APICALL
      |     elseif ~isempty(regexp([trg_port_name_spltd{1} '_' trg_port_name_spltd{2} '_' ],'^DataServices_DCM_|^RoutineServices_DCM_','once'))||...
      |             ~isempty(regexp(trg_port_name_spltd{1},'^Dcm$','once'))
      |         TaskRate = '_dcmcb';
      |         
      |     %checking if this block is used under the function call trigger
      |     %starting with "Com" and then giving an error message
      |     %this is applicable only for APICALL
      |     elseif ~isempty(regexp(trg_port_name_spltd{1},'^Com$','once'))
      |         msg = sprintf(['\n','The Supplier call block "' Thisblk '" should not be present within APICALLs having function call trigger as "Com"']);
      |         errordlg(msg);
      |         return;
      |     end
      | end
      | 
      | DataName = ['Supplier_call_esti_ti_lpos2_2sl' TaskRate];%the variable name that should be given to DataStoreRead block 
      | set_param([Thisblk '/DataStoreRead'],'DataStoreName',DataName);%Setting the DataStoreName of DataStoreRead block
      | 
      | %other settings done to this variable name
      | structVxx=Simulink.Signal;
      | structVxx.Dimensions=1;
      | structVxx.DimensionsMode='Fixed';
      | structVxx.DataType='single';
      | structVxx.Complexity='real';
      | structVxx.SamplingMode='Sample based';
      | structVxx.SampleTime=-1;
      | assignin('base',DataName,structVxx);
      settings: AttributesFormatString=%<MaskType>  RTWSystemCode=Nonreusable function  RTWFcnNameOpts=User specified
      mask Help:
      | eval('path_lib=fileparts(which(''AEMS_Standard_Library''));');
      | mskblk=get_param(gcbh,'MaskType');
      | doc_path = [path_lib '\Help\',mskblk,'.pdf'];
      | eval('open(doc_path)');
  AEMS_SUPPLIER_CALL_ESTI_TI_LPOS2_3SL : Subsystem  Tag=[LIB]  TreatAsAtomicUnit=on  RTWFcnName=SUPPLIER_CALL_Esti_ti_lpos2_3sl  mask(AEMS_SUPPLIER_CALL_ESTI_TI_LPOS2_3SL){}
      mask help:
      | Estimation of time of injection, depending on rail pressure, on fuel quantity and of fuel density
      |
      | This block is to call Supplier call API.
      mask init:
      | Thisblk = gcb;
      | model_type_pos = strsplit(Thisblk,'/');%to split all the layer paths in order to get the runnable path
      | runnable_path = [bdroot '/' model_type_pos{2}];%to get the runnable or AIPCALL path
      | trg_port_name = get_param(find_system(runnable_path,'BlockType','TriggerPort'),'Name');%to get the function call trigger name
      | TaskRate = '';%the raster suffix is stored in the parameter 
      | 
      | if ~isempty(trg_port_name)
      |     trg_port_name_spltd = strsplit(trg_port_name{1},'_');%splitting is done in order to get the raster and its type(Sched or Event)
      |     
      |     % checking for rasters of type Sched or Event especially occuring in
      |     % runnables
      |     if ~isempty(regexp(trg_port_name_spltd{1},'^Sched|^Event','once')) 
      |         TaskRate = ['_' regexprep(trg_port_name_spltd{1},'Sched|Event','','once')];
      |         
      |     %checking if the raster is dcmcb and this is applicable only for
      |     %APICALL
      |     elseif ~isempty(regexp([trg_port_name_spltd{1} '_' trg_port_name_spltd{2} '_' ],'^DataServices_DCM_|^RoutineServices_DCM_','once'))||...
      |             ~isempty(regexp(trg_port_name_spltd{1},'^Dcm$','once'))
      |         TaskRate = '_dcmcb';
      |         
      |     %checking if this block is used under the function call trigger
      |     %starting with "Com" and then giving an error message
      |     %this is applicable only for APICALL
      |     elseif ~isempty(regexp(trg_port_name_spltd{1},'^Com$','once'))
      |         msg = sprintf(['\n','The Supplier call block "' Thisblk '" should not be present within APICALLs having function call trigger as "Com"']);
      |         errordlg(msg);
      |         return;
      |     end
      | end
      | 
      | DataName = ['Supplier_call_esti_ti_lpos2_3sl' TaskRate];%the variable name that should be given to DataStoreRead block 
      | set_param([Thisblk '/DataStoreRead'],'DataStoreName',DataName);%Setting the DataStoreName of DataStoreRead block
      | 
      | %other settings done to this variable name
      | structVxx=Simulink.Signal;
      | structVxx.Dimensions=1;
      | structVxx.DimensionsMode='Fixed';
      | structVxx.DataType='single';
      | structVxx.Complexity='real';
      | structVxx.SamplingMode='Sample based';
      | structVxx.SampleTime=-1;
      | assignin('base',DataName,structVxx);
      settings: AttributesFormatString=%<MaskType>  RTWSystemCode=Nonreusable function  RTWFcnNameOpts=User specified
      mask Help:
      | eval('path_lib=fileparts(which(''AEMS_Standard_Library''));');
      | mskblk=get_param(gcbh,'MaskType');
      | doc_path = [path_lib '\Help\',mskblk,'.pdf'];
      | eval('open(doc_path)');
  AEMS_SUPPLIER_CALL_ESTI_TI_LPOS2_4SL : Subsystem  Tag=[LIB]  TreatAsAtomicUnit=on  RTWFcnName=SUPPLIER_CALL_Esti_ti_lpos2_4sl  mask(AEMS_SUPPLIER_CALL_ESTI_TI_LPOS2_4SL){}
      mask help:
      | Estimation of time of injection, depending on rail pressure, on fuel quantity and of fuel density
      |
      | This block is to call Supplier call API.
      mask init:
      | Thisblk = gcb;
      | model_type_pos = strsplit(Thisblk,'/');%to split all the layer paths in order to get the runnable path
      | runnable_path = [bdroot '/' model_type_pos{2}];%to get the runnable or AIPCALL path
      | trg_port_name = get_param(find_system(runnable_path,'BlockType','TriggerPort'),'Name');%to get the function call trigger name
      | TaskRate = '';%the raster suffix is stored in the parameter 
      | 
      | if ~isempty(trg_port_name)
      |     trg_port_name_spltd = strsplit(trg_port_name{1},'_');%splitting is done in order to get the raster and its type(Sched or Event)
      |     
      |     % checking for rasters of type Sched or Event especially occuring in
      |     % runnables
      |     if ~isempty(regexp(trg_port_name_spltd{1},'^Sched|^Event','once')) 
      |         TaskRate = ['_' regexprep(trg_port_name_spltd{1},'Sched|Event','','once')];
      |         
      |     %checking if the raster is dcmcb and this is applicable only for
      |     %APICALL
      |     elseif ~isempty(regexp([trg_port_name_spltd{1} '_' trg_port_name_spltd{2} '_' ],'^DataServices_DCM_|^RoutineServices_DCM_','once'))||...
      |             ~isempty(regexp(trg_port_name_spltd{1},'^Dcm$','once'))
      |         TaskRate = '_dcmcb';
      |         
      |     %checking if this block is used under the function call trigger
      |     %starting with "Com" and then giving an error message
      |     %this is applicable only for APICALL
      |     elseif ~isempty(regexp(trg_port_name_spltd{1},'^Com$','once'))
      |         msg = sprintf(['\n','The Supplier call block "' Thisblk '" should not be present within APICALLs having function call trigger as "Com"']);
      |         errordlg(msg);
      |         return;
      |     end
      | end
      | 
      | DataName = ['Supplier_call_esti_ti_lpos2_4sl' TaskRate];%the variable name that should be given to DataStoreRead block 
      | set_param([Thisblk '/DataStoreRead'],'DataStoreName',DataName);%Setting the DataStoreName of DataStoreRead block
      | 
      | %other settings done to this variable name
      | structVxx=Simulink.Signal;
      | structVxx.Dimensions=1;
      | structVxx.DimensionsMode='Fixed';
      | structVxx.DataType='single';
      | structVxx.Complexity='real';
      | structVxx.SamplingMode='Sample based';
      | structVxx.SampleTime=-1;
      | assignin('base',DataName,structVxx);
      settings: AttributesFormatString=%<MaskType>  RTWSystemCode=Nonreusable function  RTWFcnNameOpts=User specified
      mask Help:
      | eval('path_lib=fileparts(which(''AEMS_Standard_Library''));');
      | mskblk=get_param(gcbh,'MaskType');
      | doc_path = [path_lib '\Help\',mskblk,'.pdf'];
      | eval('open(doc_path)');
  AEMS_SUPPLIER_CALL_ESTI_TI_LPOS3_3SL : Subsystem  Tag=[LIB]  TreatAsAtomicUnit=on  RTWFcnName=SUPPLIER_CALL_Esti_ti_lpos3_3sl  mask(AEMS_SUPPLIER_CALL_ESTI_TI_LPOS3_3SL){}
      mask help:
      | Estimation of time of injection, depending on rail pressure, on fuel quantity and of fuel density
      |
      | This block is to call Supplier call API.
      mask init:
      | Thisblk = gcb;
      | model_type_pos = strsplit(Thisblk,'/');%to split all the layer paths in order to get the runnable path
      | runnable_path = [bdroot '/' model_type_pos{2}];%to get the runnable or AIPCALL path
      | trg_port_name = get_param(find_system(runnable_path,'BlockType','TriggerPort'),'Name');%to get the function call trigger name
      | TaskRate = '';%the raster suffix is stored in the parameter 
      | 
      | if ~isempty(trg_port_name)
      |     trg_port_name_spltd = strsplit(trg_port_name{1},'_');%splitting is done in order to get the raster and its type(Sched or Event)
      |     
      |     % checking for rasters of type Sched or Event especially occuring in
      |     % runnables
      |     if ~isempty(regexp(trg_port_name_spltd{1},'^Sched|^Event','once')) 
      |         TaskRate = ['_' regexprep(trg_port_name_spltd{1},'Sched|Event','','once')];
      |         
      |     %checking if the raster is dcmcb and this is applicable only for
      |     %APICALL
      |     elseif ~isempty(regexp([trg_port_name_spltd{1} '_' trg_port_name_spltd{2} '_' ],'^DataServices_DCM_|^RoutineServices_DCM_','once'))||...
      |             ~isempty(regexp(trg_port_name_spltd{1},'^Dcm$','once'))
      |         TaskRate = '_dcmcb';
      |         
      |     %checking if this block is used under the function call trigger
      |     %starting with "Com" and then giving an error message
      |     %this is applicable only for APICALL
      |     elseif ~isempty(regexp(trg_port_name_spltd{1},'^Com$','once'))
      |         msg = sprintf(['\n','The Supplier call block "' Thisblk '" should not be present within APICALLs having function call trigger as "Com"']);
      |         errordlg(msg);
      |         return;
      |     end
      | end
      | 
      | DataName = ['Supplier_call_esti_ti_lpos3_3sl' TaskRate];%the variable name that should be given to DataStoreRead block 
      | set_param([Thisblk '/DataStoreRead'],'DataStoreName',DataName);%Setting the DataStoreName of DataStoreRead block
      | 
      | %other settings done to this variable name
      | structVxx=Simulink.Signal;
      | structVxx.Dimensions=1;
      | structVxx.DimensionsMode='Fixed';
      | structVxx.DataType='single';
      | structVxx.Complexity='real';
      | structVxx.SamplingMode='Sample based';
      | structVxx.SampleTime=-1;
      | assignin('base',DataName,structVxx);
      settings: AttributesFormatString=%<MaskType>  RTWSystemCode=Nonreusable function  RTWFcnNameOpts=User specified
      mask Help:
      | eval('path_lib=fileparts(which(''AEMS_Standard_Library''));');
      | mskblk=get_param(gcbh,'MaskType');
      | doc_path = [path_lib '\Help\',mskblk,'.pdf'];
      | eval('open(doc_path)');
  AEMS_SUPPLIER_CALL_ESTI_TI_LPOS3_4SL : Subsystem  Tag=[LIB]  TreatAsAtomicUnit=on  RTWFcnName=SUPPLIER_CALL_Esti_ti_lpos3_4sl  mask(AEMS_SUPPLIER_CALL_ESTI_TI_LPOS3_4SL){}
      mask help:
      | Estimation of time of injection, depending on rail pressure, on fuel quantity and of fuel density
      |
      | This block is to call Supplier call API.
      mask init:
      | Thisblk = gcb;
      | model_type_pos = strsplit(Thisblk,'/');%to split all the layer paths in order to get the runnable path
      | runnable_path = [bdroot '/' model_type_pos{2}];%to get the runnable or AIPCALL path
      | trg_port_name = get_param(find_system(runnable_path,'BlockType','TriggerPort'),'Name');%to get the function call trigger name
      | TaskRate = '';%the raster suffix is stored in the parameter 
      | 
      | if ~isempty(trg_port_name)
      |     trg_port_name_spltd = strsplit(trg_port_name{1},'_');%splitting is done in order to get the raster and its type(Sched or Event)
      |     
      |     % checking for rasters of type Sched or Event especially occuring in
      |     % runnables
      |     if ~isempty(regexp(trg_port_name_spltd{1},'^Sched|^Event','once')) 
      |         TaskRate = ['_' regexprep(trg_port_name_spltd{1},'Sched|Event','','once')];
      |         
      |     %checking if the raster is dcmcb and this is applicable only for
      |     %APICALL
      |     elseif ~isempty(regexp([trg_port_name_spltd{1} '_' trg_port_name_spltd{2} '_' ],'^DataServices_DCM_|^RoutineServices_DCM_','once'))||...
      |             ~isempty(regexp(trg_port_name_spltd{1},'^Dcm$','once'))
      |         TaskRate = '_dcmcb';
      |         
      |     %checking if this block is used under the function call trigger
      |     %starting with "Com" and then giving an error message
      |     %this is applicable only for APICALL
      |     elseif ~isempty(regexp(trg_port_name_spltd{1},'^Com$','once'))
      |         msg = sprintf(['\n','The Supplier call block "' Thisblk '" should not be present within APICALLs having function call trigger as "Com"']);
      |         errordlg(msg);
      |         return;
      |     end
      | end
      | 
      | DataName = ['Supplier_call_esti_ti_lpos3_4sl' TaskRate];%the variable name that should be given to DataStoreRead block 
      | set_param([Thisblk '/DataStoreRead'],'DataStoreName',DataName);%Setting the DataStoreName of DataStoreRead block
      | 
      | %other settings done to this variable name
      | structVxx=Simulink.Signal;
      | structVxx.Dimensions=1;
      | structVxx.DimensionsMode='Fixed';
      | structVxx.DataType='single';
      | structVxx.Complexity='real';
      | structVxx.SamplingMode='Sample based';
      | structVxx.SampleTime=-1;
      | assignin('base',DataName,structVxx);
      settings: AttributesFormatString=%<MaskType>  RTWSystemCode=Nonreusable function  RTWFcnNameOpts=User specified
      mask Help:
      | eval('path_lib=fileparts(which(''AEMS_Standard_Library''));');
      | mskblk=get_param(gcbh,'MaskType');
      | doc_path = [path_lib '\Help\',mskblk,'.pdf'];
      | eval('open(doc_path)');
  AEMS_SUPPLIER_CALL_ESTI_TI_LPOS4_4SL : Subsystem  Tag=[LIB]  TreatAsAtomicUnit=on  RTWFcnName=SUPPLIER_CALL_Esti_ti_lpos4_4sl  mask(AEMS_SUPPLIER_CALL_ESTI_TI_LPOS4_4SL){}
      mask help:
      | Estimation of time of injection, depending on rail pressure, on fuel quantity and of fuel density
      |
      | This block is to call Supplier call API.
      mask init:
      | Thisblk = gcb;
      | model_type_pos = strsplit(Thisblk,'/');%to split all the layer paths in order to get the runnable path
      | runnable_path = [bdroot '/' model_type_pos{2}];%to get the runnable or AIPCALL path
      | trg_port_name = get_param(find_system(runnable_path,'BlockType','TriggerPort'),'Name');%to get the function call trigger name
      | TaskRate = '';%the raster suffix is stored in the parameter 
      | 
      | if ~isempty(trg_port_name)
      |     trg_port_name_spltd = strsplit(trg_port_name{1},'_');%splitting is done in order to get the raster and its type(Sched or Event)
      |     
      |     % checking for rasters of type Sched or Event especially occuring in
      |     % runnables
      |     if ~isempty(regexp(trg_port_name_spltd{1},'^Sched|^Event','once')) 
      |         TaskRate = ['_' regexprep(trg_port_name_spltd{1},'Sched|Event','','once')];
      |         
      |     %checking if the raster is dcmcb and this is applicable only for
      |     %APICALL
      |     elseif ~isempty(regexp([trg_port_name_spltd{1} '_' trg_port_name_spltd{2} '_' ],'^DataServices_DCM_|^RoutineServices_DCM_','once'))||...
      |             ~isempty(regexp(trg_port_name_spltd{1},'^Dcm$','once'))
      |         TaskRate = '_dcmcb';
      |         
      |     %checking if this block is used under the function call trigger
      |     %starting with "Com" and then giving an error message
      |     %this is applicable only for APICALL
      |     elseif ~isempty(regexp(trg_port_name_spltd{1},'^Com$','once'))
      |         msg = sprintf(['\n','The Supplier call block "' Thisblk '" should not be present within APICALLs having function call trigger as "Com"']);
      |         errordlg(msg);
      |         return;
      |     end
      | end
      | 
      | DataName = ['Supplier_call_esti_ti_lpos4_4sl' TaskRate];%the variable name that should be given to DataStoreRead block 
      | set_param([Thisblk '/DataStoreRead'],'DataStoreName',DataName);%Setting the DataStoreName of DataStoreRead block
      | 
      | %other settings done to this variable name
      | structVxx=Simulink.Signal;
      | structVxx.Dimensions=1;
      | structVxx.DimensionsMode='Fixed';
      | structVxx.DataType='single';
      | structVxx.Complexity='real';
      | structVxx.SamplingMode='Sample based';
      | structVxx.SampleTime=-1;
      | assignin('base',DataName,structVxx);
      settings: AttributesFormatString=%<MaskType>  RTWSystemCode=Nonreusable function  RTWFcnNameOpts=User specified
      mask Help:
      | eval('path_lib=fileparts(which(''AEMS_Standard_Library''));');
      | mskblk=get_param(gcbh,'MaskType');
      | doc_path = [path_lib '\Help\',mskblk,'.pdf'];
      | eval('open(doc_path)');
  AEMS_SUPPLIER_CALL_ESTI_TI_MAIN : Subsystem  Tag=[LIB]  TreatAsAtomicUnit=on  RTWFcnName=SUPPLIER_CALL_Esti_ti_main  mask(AEMS_SUPPLIER_CALL_ESTI_TI_MAIN){}
      mask help:
      | Estimation of time of injection, depending on rail pressure, on fuel quantity and of fuel density
      |
      | This block is to call Supplier call API.
      mask init:
      | Thisblk = gcb;
      | model_type_pos = strsplit(Thisblk,'/');%to split all the layer paths in order to get the runnable path
      | runnable_path = [bdroot '/' model_type_pos{2}];%to get the runnable or AIPCALL path
      | trg_port_name = get_param(find_system(runnable_path,'BlockType','TriggerPort'),'Name');%to get the function call trigger name
      | TaskRate = '';%the raster suffix is stored in the parameter 
      | 
      | if ~isempty(trg_port_name)
      |     trg_port_name_spltd = strsplit(trg_port_name{1},'_');%splitting is done in order to get the raster and its type(Sched or Event)
      |     
      |     % checking for rasters of type Sched or Event especially occuring in
      |     % runnables
      |     if ~isempty(regexp(trg_port_name_spltd{1},'^Sched|^Event','once')) 
      |         TaskRate = ['_' regexprep(trg_port_name_spltd{1},'Sched|Event','','once')];
      |         
      |     %checking if the raster is dcmcb and this is applicable only for
      |     %APICALL
      |     elseif ~isempty(regexp([trg_port_name_spltd{1} '_' trg_port_name_spltd{2} '_' ],'^DataServices_DCM_|^RoutineServices_DCM_','once'))||...
      |             ~isempty(regexp(trg_port_name_spltd{1},'^Dcm$','once'))
      |         TaskRate = '_dcmcb';
      |         
      |     %checking if this block is used under the function call trigger
      |     %starting with "Com" and then giving an error message
      |     %this is applicable only for APICALL
      |     elseif ~isempty(regexp(trg_port_name_spltd{1},'^Com$','once'))
      |         msg = sprintf(['\n','The Supplier call block "' Thisblk '" should not be present within APICALLs having function call trigger as "Com"']);
      |         errordlg(msg);
      |         return;
      |     end
      | end
      | 
      | DataName = ['Supplier_call_esti_ti_main' TaskRate];%the variable name that should be given to DataStoreRead block 
      | set_param([Thisblk '/DataStoreRead'],'DataStoreName',DataName);%Setting the DataStoreName of DataStoreRead block
      | 
      | %other settings done to this variable name
      | structVxx=Simulink.Signal;
      | structVxx.Dimensions=1;
      | structVxx.DimensionsMode='Fixed';
      | structVxx.DataType='single';
      | structVxx.Complexity='real';
      | structVxx.SamplingMode='Sample based';
      | structVxx.SampleTime=-1;
      | assignin('base',DataName,structVxx);
      settings: AttributesFormatString=%<MaskType>  RTWSystemCode=Nonreusable function  RTWFcnNameOpts=User specified
      mask Help:
      | eval('path_lib=fileparts(which(''AEMS_Standard_Library''));');
      | mskblk=get_param(gcbh,'MaskType');
      | doc_path = [path_lib '\Help\',mskblk,'.pdf'];
      | eval('open(doc_path)');
  AEMS_SUPPLIER_CALL_ESTI_TI_MAIN_AFTR : Subsystem  Tag=[LIB]  TreatAsAtomicUnit=on  RTWFcnName=SUPPLIER_CALL_Esti_ti_main_aftr  mask(AEMS_SUPPLIER_CALL_ESTI_TI_MAIN_AFTR){}
      mask help:
      | Estimation of time of injection, depending on rail pressure, on fuel quantity and of fuel density
      |
      | This block is to call Supplier call API.
      mask init:
      | Thisblk = gcb;
      | model_type_pos = strsplit(Thisblk,'/');%to split all the layer paths in order to get the runnable path
      | runnable_path = [bdroot '/' model_type_pos{2}];%to get the runnable or AIPCALL path
      | trg_port_name = get_param(find_system(runnable_path,'BlockType','TriggerPort'),'Name');%to get the function call trigger name
      | TaskRate = '';%the raster suffix is stored in the parameter 
      | 
      | if ~isempty(trg_port_name)
      |     trg_port_name_spltd = strsplit(trg_port_name{1},'_');%splitting is done in order to get the raster and its type(Sched or Event)
      |     
      |     % checking for rasters of type Sched or Event especially occuring in
      |     % runnables
      |     if ~isempty(regexp(trg_port_name_spltd{1},'^Sched|^Event','once')) 
      |         TaskRate = ['_' regexprep(trg_port_name_spltd{1},'Sched|Event','','once')];
      |         
      |     %checking if the raster is dcmcb and this is applicable only for
      |     %APICALL
      |     elseif ~isempty(regexp([trg_port_name_spltd{1} '_' trg_port_name_spltd{2} '_' ],'^DataServices_DCM_|^RoutineServices_DCM_','once'))||...
      |             ~isempty(regexp(trg_port_name_spltd{1},'^Dcm$','once'))
      |         TaskRate = '_dcmcb';
      |         
      |     %checking if this block is used under the function call trigger
      |     %starting with "Com" and then giving an error message
      |     %this is applicable only for APICALL
      |     elseif ~isempty(regexp(trg_port_name_spltd{1},'^Com$','once'))
      |         msg = sprintf(['\n','The Supplier call block "' Thisblk '" should not be present within APICALLs having function call trigger as "Com"']);
      |         errordlg(msg);
      |         return;
      |     end
      | end
      | 
      | DataName = ['Supplier_call_esti_ti_main_aftr' TaskRate];%the variable name that should be given to DataStoreRead block 
      | set_param([Thisblk '/DataStoreRead'],'DataStoreName',DataName);%Setting the DataStoreName of DataStoreRead block
      | 
      | %other settings done to this variable name
      | structVxx=Simulink.Signal;
      | structVxx.Dimensions=1;
      | structVxx.DimensionsMode='Fixed';
      | structVxx.DataType='single';
      | structVxx.Complexity='real';
      | structVxx.SamplingMode='Sample based';
      | structVxx.SampleTime=-1;
      | assignin('base',DataName,structVxx);
      settings: AttributesFormatString=%<MaskType>  RTWSystemCode=Nonreusable function  RTWFcnNameOpts=User specified
      mask Help:
      | eval('path_lib=fileparts(which(''AEMS_Standard_Library''));');
      | mskblk=get_param(gcbh,'MaskType');
      | doc_path = [path_lib '\Help\',mskblk,'.pdf'];
      | eval('open(doc_path)');
  AEMS_SUPPLIER_CALL_ESTI_TI_MAIN_POST : Subsystem  Tag=[LIB]  TreatAsAtomicUnit=on  RTWFcnName=SUPPLIER_CALL_Esti_ti_main_post  mask(AEMS_SUPPLIER_CALL_ESTI_TI_MAIN_POST){}
      mask help:
      | Estimation of time of injection, depending on rail pressure, on fuel quantity and of fuel density
      |
      | This block is to call Supplier call API.
      mask init:
      | Thisblk = gcb;
      | model_type_pos = strsplit(Thisblk,'/');%to split all the layer paths in order to get the runnable path
      | runnable_path = [bdroot '/' model_type_pos{2}];%to get the runnable or AIPCALL path
      | trg_port_name = get_param(find_system(runnable_path,'BlockType','TriggerPort'),'Name');%to get the function call trigger name
      | TaskRate = '';%the raster suffix is stored in the parameter 
      | 
      | if ~isempty(trg_port_name)
      |     trg_port_name_spltd = strsplit(trg_port_name{1},'_');%splitting is done in order to get the raster and its type(Sched or Event)
      |     
      |     % checking for rasters of type Sched or Event especially occuring in
      |     % runnables
      |     if ~isempty(regexp(trg_port_name_spltd{1},'^Sched|^Event','once')) 
      |         TaskRate = ['_' regexprep(trg_port_name_spltd{1},'Sched|Event','','once')];
      |         
      |     %checking if the raster is dcmcb and this is applicable only for
      |     %APICALL
      |     elseif ~isempty(regexp([trg_port_name_spltd{1} '_' trg_port_name_spltd{2} '_' ],'^DataServices_DCM_|^RoutineServices_DCM_','once'))||...
      |             ~isempty(regexp(trg_port_name_spltd{1},'^Dcm$','once'))
      |         TaskRate = '_dcmcb';
      |         
      |     %checking if this block is used under the function call trigger
      |     %starting with "Com" and then giving an error message
      |     %this is applicable only for APICALL
      |     elseif ~isempty(regexp(trg_port_name_spltd{1},'^Com$','once'))
      |         msg = sprintf(['\n','The Supplier call block "' Thisblk '" should not be present within APICALLs having function call trigger as "Com"']);
      |         errordlg(msg);
      |         return;
      |     end
      | end
      | 
      | DataName = ['Supplier_call_esti_ti_main_post' TaskRate];%the variable name that should be given to DataStoreRead block 
      | set_param([Thisblk '/DataStoreRead'],'DataStoreName',DataName);%Setting the DataStoreName of DataStoreRead block
      | 
      | %other settings done to this variable name
      | structVxx=Simulink.Signal;
      | structVxx.Dimensions=1;
      | structVxx.DimensionsMode='Fixed';
      | structVxx.DataType='single';
      | structVxx.Complexity='real';
      | structVxx.SamplingMode='Sample based';
      | structVxx.SampleTime=-1;
      | assignin('base',DataName,structVxx);
      settings: AttributesFormatString=%<MaskType>  RTWSystemCode=Nonreusable function  RTWFcnNameOpts=User specified
      mask Help:
      | eval('path_lib=fileparts(which(''AEMS_Standard_Library''));');
      | mskblk=get_param(gcbh,'MaskType');
      | doc_path = [path_lib '\Help\',mskblk,'.pdf'];
      | eval('open(doc_path)');
  AEMS_SUPPLIER_CALL_ESTI_TI_PINJ1 : Subsystem  Tag=[LIB]  TreatAsAtomicUnit=on  RTWFcnName=SUPPLIER_CALL_Esti_ti_pinj1  mask(AEMS_SUPPLIER_CALL_ESTI_TI_PINJ1){}
      mask help:
      | Estimation of time of injection
      |
      | This block is to call Supplier call API.
      mask init:
      | Thisblk = gcb;
      | model_type_pos = strsplit(Thisblk,'/');%to split all the layer paths in order to get the runnable path
      | runnable_path = [bdroot '/' model_type_pos{2}];%to get the runnable or AIPCALL path
      | trg_port_name = get_param(find_system(runnable_path,'BlockType','TriggerPort'),'Name');%to get the function call trigger name
      | TaskRate = '';%the raster suffix is stored in the parameter 
      | 
      | if ~isempty(trg_port_name)
      |     trg_port_name_spltd = strsplit(trg_port_name{1},'_');%splitting is done in order to get the raster and its type(Sched or Event)
      |     
      |     % checking for rasters of type Sched or Event especially occuring in
      |     % runnables
      |     if ~isempty(regexp(trg_port_name_spltd{1},'^Sched|^Event','once')) 
      |         TaskRate = ['_' regexprep(trg_port_name_spltd{1},'Sched|Event','','once')];
      |         
      |     %checking if the raster is dcmcb and this is applicable only for
      |     %APICALL
      |     elseif ~isempty(regexp([trg_port_name_spltd{1} '_' trg_port_name_spltd{2} '_' ],'^DataServices_DCM_|^RoutineServices_DCM_','once'))||...
      |             ~isempty(regexp(trg_port_name_spltd{1},'^Dcm$','once'))
      |         TaskRate = '_dcmcb';
      |         
      |     %checking if this block is used under the function call trigger
      |     %starting with "Com" and then giving an error message
      |     %this is applicable only for APICALL
      |     elseif ~isempty(regexp(trg_port_name_spltd{1},'^Com$','once'))
      |         msg = sprintf(['\n','The Supplier call block "' Thisblk '" should not be present within APICALLs having function call trigger as "Com"']);
      |         errordlg(msg);
      |         return;
      |     end
      | end
      | 
      | DataName = ['Supplier_call_esti_ti_pinj1' TaskRate];%the variable name that should be given to DataStoreRead block 
      | set_param([Thisblk '/DataStoreRead'],'DataStoreName',DataName);%Setting the DataStoreName of DataStoreRead block
      | 
      | %other settings done to this variable name
      | structVxx=Simulink.Signal;
      | structVxx.Dimensions=1;
      | structVxx.DimensionsMode='Fixed';
      | structVxx.DataType='single';
      | structVxx.Complexity='real';
      | structVxx.SamplingMode='Sample based';
      | structVxx.SampleTime=-1;
      | assignin('base',DataName,structVxx);
      settings: AttributesFormatString=%<MaskType>  RTWSystemCode=Nonreusable function  RTWFcnNameOpts=User specified
      mask Help:
      | eval('path_lib=fileparts(which(''AEMS_Standard_Library''));');
      | mskblk=get_param(gcbh,'MaskType');
      | doc_path = [path_lib '\Help\',mskblk,'.pdf'];
      | eval('open(doc_path)');
  AEMS_SUPPLIER_CALL_ESTI_TI_PINJ2 : Subsystem  Tag=[LIB]  TreatAsAtomicUnit=on  RTWFcnName=SUPPLIER_CALL_Esti_ti_pinj2  mask(AEMS_SUPPLIER_CALL_ESTI_TI_PINJ2){}
      mask help:
      | Estimation of time of injection
      |
      | This block is to call Supplier call API.
      mask init:
      | Thisblk = gcb;
      | model_type_pos = strsplit(Thisblk,'/');%to split all the layer paths in order to get the runnable path
      | runnable_path = [bdroot '/' model_type_pos{2}];%to get the runnable or AIPCALL path
      | trg_port_name = get_param(find_system(runnable_path,'BlockType','TriggerPort'),'Name');%to get the function call trigger name
      | TaskRate = '';%the raster suffix is stored in the parameter 
      | 
      | if ~isempty(trg_port_name)
      |     trg_port_name_spltd = strsplit(trg_port_name{1},'_');%splitting is done in order to get the raster and its type(Sched or Event)
      |     
      |     % checking for rasters of type Sched or Event especially occuring in
      |     % runnables
      |     if ~isempty(regexp(trg_port_name_spltd{1},'^Sched|^Event','once')) 
      |         TaskRate = ['_' regexprep(trg_port_name_spltd{1},'Sched|Event','','once')];
      |         
      |     %checking if the raster is dcmcb and this is applicable only for
      |     %APICALL
      |     elseif ~isempty(regexp([trg_port_name_spltd{1} '_' trg_port_name_spltd{2} '_' ],'^DataServices_DCM_|^RoutineServices_DCM_','once'))||...
      |             ~isempty(regexp(trg_port_name_spltd{1},'^Dcm$','once'))
      |         TaskRate = '_dcmcb';
      |         
      |     %checking if this block is used under the function call trigger
      |     %starting with "Com" and then giving an error message
      |     %this is applicable only for APICALL
      |     elseif ~isempty(regexp(trg_port_name_spltd{1},'^Com$','once'))
      |         msg = sprintf(['\n','The Supplier call block "' Thisblk '" should not be present within APICALLs having function call trigger as "Com"']);
      |         errordlg(msg);
      |         return;
      |     end
      | end
      | 
      | DataName = ['Supplier_call_esti_ti_pinj2' TaskRate];%the variable name that should be given to DataStoreRead block 
      | set_param([Thisblk '/DataStoreRead'],'DataStoreName',DataName);%Setting the DataStoreName of DataStoreRead block
      | 
      | %other settings done to this variable name
      | structVxx=Simulink.Signal;
      | structVxx.Dimensions=1;
      | structVxx.DimensionsMode='Fixed';
      | structVxx.DataType='single';
      | structVxx.Complexity='real';
      | structVxx.SamplingMode='Sample based';
      | structVxx.SampleTime=-1;
      | assignin('base',DataName,structVxx);
      settings: AttributesFormatString=%<MaskType>  RTWSystemCode=Nonreusable function  RTWFcnNameOpts=User specified
      mask Help:
      | eval('path_lib=fileparts(which(''AEMS_Standard_Library''));');
      | mskblk=get_param(gcbh,'MaskType');
      | doc_path = [path_lib '\Help\',mskblk,'.pdf'];
      | eval('open(doc_path)');
  AEMS_SUPPLIER_CALL_ESTI_TI_PINJ3 : Subsystem  Tag=[LIB]  TreatAsAtomicUnit=on  RTWFcnName=SUPPLIER_CALL_Esti_ti_pinj3  mask(AEMS_SUPPLIER_CALL_ESTI_TI_PINJ3){}
      mask help:
      | Estimation of time of injection
      |
      | This block is to call Supplier call API.
      mask init:
      | Thisblk = gcb;
      | model_type_pos = strsplit(Thisblk,'/');%to split all the layer paths in order to get the runnable path
      | runnable_path = [bdroot '/' model_type_pos{2}];%to get the runnable or AIPCALL path
      | trg_port_name = get_param(find_system(runnable_path,'BlockType','TriggerPort'),'Name');%to get the function call trigger name
      | TaskRate = '';%the raster suffix is stored in the parameter 
      | 
      | if ~isempty(trg_port_name)
      |     trg_port_name_spltd = strsplit(trg_port_name{1},'_');%splitting is done in order to get the raster and its type(Sched or Event)
      |     
      |     % checking for rasters of type Sched or Event especially occuring in
      |     % runnables
      |     if ~isempty(regexp(trg_port_name_spltd{1},'^Sched|^Event','once')) 
      |         TaskRate = ['_' regexprep(trg_port_name_spltd{1},'Sched|Event','','once')];
      |         
      |     %checking if the raster is dcmcb and this is applicable only for
      |     %APICALL
      |     elseif ~isempty(regexp([trg_port_name_spltd{1} '_' trg_port_name_spltd{2} '_' ],'^DataServices_DCM_|^RoutineServices_DCM_','once'))||...
      |             ~isempty(regexp(trg_port_name_spltd{1},'^Dcm$','once'))
      |         TaskRate = '_dcmcb';
      |         
      |     %checking if this block is used under the function call trigger
      |     %starting with "Com" and then giving an error message
      |     %this is applicable only for APICALL
      |     elseif ~isempty(regexp(trg_port_name_spltd{1},'^Com$','once'))
      |         msg = sprintf(['\n','The Supplier call block "' Thisblk '" should not be present within APICALLs having function call trigger as "Com"']);
      |         errordlg(msg);
      |         return;
      |     end
      | end
      | 
      | DataName = ['Supplier_call_esti_ti_pinj3' TaskRate];%the variable name that should be given to DataStoreRead block 
      | set_param([Thisblk '/DataStoreRead'],'DataStoreName',DataName);%Setting the DataStoreName of DataStoreRead block
      | 
      | %other settings done to this variable name
      | structVxx=Simulink.Signal;
      | structVxx.Dimensions=1;
      | structVxx.DimensionsMode='Fixed';
      | structVxx.DataType='single';
      | structVxx.Complexity='real';
      | structVxx.SamplingMode='Sample based';
      | structVxx.SampleTime=-1;
      | assignin('base',DataName,structVxx);
      settings: AttributesFormatString=%<MaskType>  RTWSystemCode=Nonreusable function  RTWFcnNameOpts=User specified  RTWFileNameOpts=User specified
      mask Help:
      | eval('path_lib=fileparts(which(''AEMS_Standard_Library''));');
      | mskblk=get_param(gcbh,'MaskType');
      | doc_path = [path_lib '\Help\',mskblk,'.pdf'];
      | eval('open(doc_path)');
  AEMS_SUPPLIER_CALL_ESTI_TI_PINJ4 : Subsystem  Tag=[LIB]  TreatAsAtomicUnit=on  RTWFcnName=SUPPLIER_CALL_Esti_ti_pinj4  mask(AEMS_SUPPLIER_CALL_ESTI_TI_PINJ4){}
      mask help:
      | Estimation of time of injection
      |
      | This block is to call Supplier call API.
      mask init:
      | Thisblk = gcb;
      | model_type_pos = strsplit(Thisblk,'/');%to split all the layer paths in order to get the runnable path
      | runnable_path = [bdroot '/' model_type_pos{2}];%to get the runnable or AIPCALL path
      | trg_port_name = get_param(find_system(runnable_path,'BlockType','TriggerPort'),'Name');%to get the function call trigger name
      | TaskRate = '';%the raster suffix is stored in the parameter 
      | 
      | if ~isempty(trg_port_name)
      |     trg_port_name_spltd = strsplit(trg_port_name{1},'_');%splitting is done in order to get the raster and its type(Sched or Event)
      |     
      |     % checking for rasters of type Sched or Event especially occuring in
      |     % runnables
      |     if ~isempty(regexp(trg_port_name_spltd{1},'^Sched|^Event','once')) 
      |         TaskRate = ['_' regexprep(trg_port_name_spltd{1},'Sched|Event','','once')];
      |         
      |     %checking if the raster is dcmcb and this is applicable only for
      |     %APICALL
      |     elseif ~isempty(regexp([trg_port_name_spltd{1} '_' trg_port_name_spltd{2} '_' ],'^DataServices_DCM_|^RoutineServices_DCM_','once'))||...
      |             ~isempty(regexp(trg_port_name_spltd{1},'^Dcm$','once'))
      |         TaskRate = '_dcmcb';
      |         
      |     %checking if this block is used under the function call trigger
      |     %starting with "Com" and then giving an error message
      |     %this is applicable only for APICALL
      |     elseif ~isempty(regexp(trg_port_name_spltd{1},'^Com$','once'))
      |         msg = sprintf(['\n','The Supplier call block "' Thisblk '" should not be present within APICALLs having function call trigger as "Com"']);
      |         errordlg(msg);
      |         return;
      |     end
      | end
      | 
      | DataName = ['Supplier_call_esti_ti_pinj4' TaskRate];%the variable name that should be given to DataStoreRead block 
      | set_param([Thisblk '/DataStoreRead'],'DataStoreName',DataName);%Setting the DataStoreName of DataStoreRead block
      | 
      | %other settings done to this variable name
      | structVxx=Simulink.Signal;
      | structVxx.Dimensions=1;
      | structVxx.DimensionsMode='Fixed';
      | structVxx.DataType='single';
      | structVxx.Complexity='real';
      | structVxx.SamplingMode='Sample based';
      | structVxx.SampleTime=-1;
      | assignin('base',DataName,structVxx);
      settings: AttributesFormatString=%<MaskType>  RTWSystemCode=Nonreusable function  RTWFcnNameOpts=User specified  RTWFileNameOpts=User specified
      mask Help:
      | eval('path_lib=fileparts(which(''AEMS_Standard_Library''));');
      | mskblk=get_param(gcbh,'MaskType');
      | doc_path = [path_lib '\Help\',mskblk,'.pdf'];
      | eval('open(doc_path)');
  AEMS_SUPPLIER_CALL_ESTI_TI_POST : Subsystem  Tag=[LIB]  TreatAsAtomicUnit=on  RTWFcnName=SUPPLIER_CALL_Esti_ti_post  mask(AEMS_SUPPLIER_CALL_ESTI_TI_POST){}
      mask help:
      | Estimation of time of injection, depending on rail pressure, on fuel quantity and of fuel density
      |
      | This block is to call Supplier call API.
      mask init:
      | Thisblk = gcb;
      | model_type_pos = strsplit(Thisblk,'/');%to split all the layer paths in order to get the runnable path
      | runnable_path = [bdroot '/' model_type_pos{2}];%to get the runnable or AIPCALL path
      | trg_port_name = get_param(find_system(runnable_path,'BlockType','TriggerPort'),'Name');%to get the function call trigger name
      | TaskRate = '';%the raster suffix is stored in the parameter 
      | 
      | if ~isempty(trg_port_name)
      |     trg_port_name_spltd = strsplit(trg_port_name{1},'_');%splitting is done in order to get the raster and its type(Sched or Event)
      |     
      |     % checking for rasters of type Sched or Event especially occuring in
      |     % runnables
      |     if ~isempty(regexp(trg_port_name_spltd{1},'^Sched|^Event','once')) 
      |         TaskRate = ['_' regexprep(trg_port_name_spltd{1},'Sched|Event','','once')];
      |         
      |     %checking if the raster is dcmcb and this is applicable only for
      |     %APICALL
      |     elseif ~isempty(regexp([trg_port_name_spltd{1} '_' trg_port_name_spltd{2} '_' ],'^DataServices_DCM_|^RoutineServices_DCM_','once'))||...
      |             ~isempty(regexp(trg_port_name_spltd{1},'^Dcm$','once'))
      |         TaskRate = '_dcmcb';
      |         
      |     %checking if this block is used under the function call trigger
      |     %starting with "Com" and then giving an error message
      |     %this is applicable only for APICALL
      |     elseif ~isempty(regexp(trg_port_name_spltd{1},'^Com$','once'))
      |         msg = sprintf(['\n','The Supplier call block "' Thisblk '" should not be present within APICALLs having function call trigger as "Com"']);
      |         errordlg(msg);
      |         return;
      |     end
      | end
      | 
      | DataName = ['Supplier_call_esti_ti_post' TaskRate];%the variable name that should be given to DataStoreRead block 
      | set_param([Thisblk '/DataStoreRead'],'DataStoreName',DataName);%Setting the DataStoreName of DataStoreRead block
      | 
      | %other settings done to this variable name
      | structVxx=Simulink.Signal;
      | structVxx.Dimensions=1;
      | structVxx.DimensionsMode='Fixed';
      | structVxx.DataType='single';
      | structVxx.Complexity='real';
      | structVxx.SamplingMode='Sample based';
      | structVxx.SampleTime=-1;
      | assignin('base',DataName,structVxx);
      settings: AttributesFormatString=%<MaskType>  RTWSystemCode=Nonreusable function  RTWFcnNameOpts=User specified
      mask Help:
      | eval('path_lib=fileparts(which(''AEMS_Standard_Library''));');
      | mskblk=get_param(gcbh,'MaskType');
      | doc_path = [path_lib '\Help\',mskblk,'.pdf'];
      | eval('open(doc_path)');
  AEMS_SUPPLIER_CALL_FIM_MAX : Subsystem  Tag=[LIB]  TreatAsAtomicUnit=on  RTWFcnName=SUPPLIER_CALL_Fim_max  mask(AEMS_SUPPLIER_CALL_FIM_MAX){}
      mask help:
      | Fuel injection minimum mass depending on rail pressure.
      |
      | This block is to call Supplier call API.
      mask init:
      | Thisblk = gcb;
      | model_type_pos = strsplit(Thisblk,'/');%to split all the layer paths in order to get the runnable path
      | runnable_path = [bdroot '/' model_type_pos{2}];%to get the runnable or AIPCALL path
      | trg_port_name = get_param(find_system(runnable_path,'BlockType','TriggerPort'),'Name');%to get the function call trigger name
      | TaskRate = '';%the raster suffix is stored in the parameter 
      | 
      | if ~isempty(trg_port_name)
      |     trg_port_name_spltd = strsplit(trg_port_name{1},'_');%splitting is done in order to get the raster and its type(Sched or Event)
      |     
      |     % checking for rasters of type Sched or Event especially occuring in
      |     % runnables
      |     if ~isempty(regexp(trg_port_name_spltd{1},'^Sched|^Event','once')) 
      |         TaskRate = ['_' regexprep(trg_port_name_spltd{1},'Sched|Event','','once')];
      |         
      |     %checking if the raster is dcmcb and this is applicable only for
      |     %APICALL
      |     elseif ~isempty(regexp([trg_port_name_spltd{1} '_' trg_port_name_spltd{2} '_' ],'^DataServices_DCM_|^RoutineServices_DCM_','once'))||...
      |             ~isempty(regexp(trg_port_name_spltd{1},'^Dcm$','once'))
      |         TaskRate = '_dcmcb';
      |         
      |     %checking if this block is used under the function call trigger
      |     %starting with "Com" and then giving an error message
      |     %this is applicable only for APICALL
      |     elseif ~isempty(regexp(trg_port_name_spltd{1},'^Com$','once'))
      |         msg = sprintf(['\n','The Supplier call block "' Thisblk '" should not be present within APICALLs having function call trigger as "Com"']);
      |         errordlg(msg);
      |         return;
      |     end
      | end
      | 
      | DataName = ['Supplier_call_fim_max' TaskRate];%the variable name that should be given to DataStoreRead block 
      | set_param([Thisblk '/DataStoreRead'],'DataStoreName',DataName);%Setting the DataStoreName of DataStoreRead block
      | 
      | %other settings done to this variable name
      | structVxx=Simulink.Signal;
      | structVxx.Dimensions=1;
      | structVxx.DimensionsMode='Fixed';
      | structVxx.DataType='single';
      | structVxx.Complexity='real';
      | structVxx.SamplingMode='Sample based';
      | structVxx.SampleTime=-1;
      | assignin('base',DataName,structVxx);
      settings: AttributesFormatString=%<MaskType>  RTWSystemCode=Nonreusable function  RTWFcnNameOpts=User specified  RTWFileNameOpts=User specified
      mask Help:
      | eval('path_lib=fileparts(which(''AEMS_Standard_Library''));');
      | mskblk=get_param(gcbh,'MaskType');
      | doc_path = [path_lib '\Help\',mskblk,'.pdf'];
      | eval('open(doc_path)');
  AEMS_SUPPLIER_CALL_FIM_MIN_AFTR : Subsystem  Tag=[LIB]  TreatAsAtomicUnit=on  RTWFcnName=SUPPLIER_CALL_Fim_min_aftr  mask(AEMS_SUPPLIER_CALL_FIM_MIN_AFTR){}
      mask help:
      | Fuel injection minimum mass depending on rail pressure.
      |
      | This block is to call Supplier call API.
      mask init:
      | Thisblk = gcb;
      | model_type_pos = strsplit(Thisblk,'/');%to split all the layer paths in order to get the runnable path
      | runnable_path = [bdroot '/' model_type_pos{2}];%to get the runnable or AIPCALL path
      | trg_port_name = get_param(find_system(runnable_path,'BlockType','TriggerPort'),'Name');%to get the function call trigger name
      | TaskRate = '';%the raster suffix is stored in the parameter 
      | 
      | if ~isempty(trg_port_name)
      |     trg_port_name_spltd = strsplit(trg_port_name{1},'_');%splitting is done in order to get the raster and its type(Sched or Event)
      |     
      |     % checking for rasters of type Sched or Event especially occuring in
      |     % runnables
      |     if ~isempty(regexp(trg_port_name_spltd{1},'^Sched|^Event','once')) 
      |         TaskRate = ['_' regexprep(trg_port_name_spltd{1},'Sched|Event','','once')];
      |         
      |     %checking if the raster is dcmcb and this is applicable only for
      |     %APICALL
      |     elseif ~isempty(regexp([trg_port_name_spltd{1} '_' trg_port_name_spltd{2} '_' ],'^DataServices_DCM_|^RoutineServices_DCM_','once'))||...
      |             ~isempty(regexp(trg_port_name_spltd{1},'^Dcm$','once'))
      |         TaskRate = '_dcmcb';
      |         
      |     %checking if this block is used under the function call trigger
      |     %starting with "Com" and then giving an error message
      |     %this is applicable only for APICALL
      |     elseif ~isempty(regexp(trg_port_name_spltd{1},'^Com$','once'))
      |         msg = sprintf(['\n','The Supplier call block "' Thisblk '" should not be present within APICALLs having function call trigger as "Com"']);
      |         errordlg(msg);
      |         return;
      |     end
      | end
      | 
      | DataName = ['Supplier_call_fim_min' TaskRate];%the variable name that should be given to DataStoreRead block 
      | set_param([Thisblk '/Data Store Read'],'DataStoreName',DataName);%Setting the DataStoreName of DataStoreRead block
      | 
      | %other settings done to this variable name
      | structVxx=Simulink.Signal;
      | structVxx.Dimensions=1;
      | structVxx.DimensionsMode='Fixed';
      | structVxx.DataType='single';
      | structVxx.Complexity='real';
      | structVxx.SamplingMode='Sample based';
      | structVxx.SampleTime=-1;
      | assignin('base',DataName,structVxx);
      settings: AttributesFormatString=%<MaskType>  RTWSystemCode=Nonreusable function  RTWFcnNameOpts=User specified
      mask Help:
      | eval('path_lib=fileparts(which(''AEMS_Standard_Library''));');
      | mskblk=get_param(gcbh,'MaskType');
      | doc_path = [path_lib '\Help\',mskblk,'.pdf'];
      | eval('open(doc_path)');
  AEMS_SUPPLIER_CALL_FIM_MIN_LPOS1 : Subsystem  Tag=[LIB]  TreatAsAtomicUnit=on  RTWFcnName=SUPPLIER_CALL_Fim_min_lpos1  mask(AEMS_SUPPLIER_CALL_FIM_MIN_LPOS1){}
      mask help:
      | Fuel injection minimum mass depending on rail pressure.
      |
      | This block is to call Supplier call API.
      mask init:
      | Thisblk = gcb;
      | model_type_pos = strsplit(Thisblk,'/');%to split all the layer paths in order to get the runnable path
      | runnable_path = [bdroot '/' model_type_pos{2}];%to get the runnable or AIPCALL path
      | trg_port_name = get_param(find_system(runnable_path,'BlockType','TriggerPort'),'Name');%to get the function call trigger name
      | TaskRate = '';%the raster suffix is stored in the parameter 
      | 
      | if ~isempty(trg_port_name)
      |     trg_port_name_spltd = strsplit(trg_port_name{1},'_');%splitting is done in order to get the raster and its type(Sched or Event)
      |     
      |     % checking for rasters of type Sched or Event especially occuring in
      |     % runnables
      |     if ~isempty(regexp(trg_port_name_spltd{1},'^Sched|^Event','once')) 
      |         TaskRate = ['_' regexprep(trg_port_name_spltd{1},'Sched|Event','','once')];
      |         
      |     %checking if the raster is dcmcb and this is applicable only for
      |     %APICALL
      |     elseif ~isempty(regexp([trg_port_name_spltd{1} '_' trg_port_name_spltd{2} '_' ],'^DataServices_DCM_|^RoutineServices_DCM_','once'))||...
      |             ~isempty(regexp(trg_port_name_spltd{1},'^Dcm$','once'))
      |         TaskRate = '_dcmcb';
      |         
      |     %checking if this block is used under the function call trigger
      |     %starting with "Com" and then giving an error message
      |     %this is applicable only for APICALL
      |     elseif ~isempty(regexp(trg_port_name_spltd{1},'^Com$','once'))
      |         msg = sprintf(['\n','The Supplier call block "' Thisblk '" should not be present within APICALLs having function call trigger as "Com"']);
      |         errordlg(msg);
      |         return;
      |     end
      | end
      | 
      | DataName = ['Supplier_call_fim_min' TaskRate];%the variable name that should be given to DataStoreRead block 
      | set_param([Thisblk '/Data Store Read'],'DataStoreName',DataName);%Setting the DataStoreName of DataStoreRead block
      | 
      | %other settings done to this variable name
      | structVxx=Simulink.Signal;
      | structVxx.Dimensions=1;
      | structVxx.DimensionsMode='Fixed';
      | structVxx.DataType='single';
      | structVxx.Complexity='real';
      | structVxx.SamplingMode='Sample based';
      | structVxx.SampleTime=-1;
      | assignin('base',DataName,structVxx);
      settings: AttributesFormatString=%<MaskType>  RTWSystemCode=Nonreusable function  RTWFcnNameOpts=User specified
      mask Help:
      | eval('path_lib=fileparts(which(''AEMS_Standard_Library''));');
      | mskblk=get_param(gcbh,'MaskType');
      | doc_path = [path_lib '\Help\',mskblk,'.pdf'];
      | eval('open(doc_path)');
  AEMS_SUPPLIER_CALL_FIM_MIN_LPOS1_2SL : Subsystem  Tag=[LIB]  TreatAsAtomicUnit=on  RTWFcnName=SUPPLIER_CALL_Fim_min_lpos1_2sl  mask(AEMS_SUPPLIER_CALL_FIM_MIN_LPOS1_2SL){}
      mask help:
      | Fuel injection minimum mass depending on rail pressure.
      |
      | This block is to call Supplier call API.
      mask init: same as AEMS_Standard_Library/SPECIFIC/AEMS_SUPPLIER_CALL_FIM_MIN_AFTR
      settings: AttributesFormatString=%<MaskType>  RTWSystemCode=Nonreusable function  RTWFcnNameOpts=User specified
      mask Help:
      | eval('path_lib=fileparts(which(''AEMS_Standard_Library''));');
      | mskblk=get_param(gcbh,'MaskType');
      | doc_path = [path_lib '\Help\',mskblk,'.pdf'];
      | eval('open(doc_path)');
  AEMS_SUPPLIER_CALL_FIM_MIN_LPOS1_3SL : Subsystem  Tag=[LIB]  TreatAsAtomicUnit=on  RTWFcnName=SUPPLIER_CALL_Fim_min_lpos1_3sl  mask(AEMS_SUPPLIER_CALL_FIM_MIN_LPOS1_3SL){}
      mask help:
      | Fuel injection minimum mass depending on rail pressure.
      |
      | This block is to call Supplier call API.
      mask init: same as AEMS_Standard_Library/SPECIFIC/AEMS_SUPPLIER_CALL_FIM_MIN_AFTR
      settings: AttributesFormatString=%<MaskType>  RTWSystemCode=Nonreusable function  RTWFcnNameOpts=User specified
      mask Help:
      | eval('path_lib=fileparts(which(''AEMS_Standard_Library''));');
      | mskblk=get_param(gcbh,'MaskType');
      | doc_path = [path_lib '\Help\',mskblk,'.pdf'];
      | eval('open(doc_path)');
  AEMS_SUPPLIER_CALL_FIM_MIN_LPOS1_4SL : Subsystem  Tag=[LIB]  TreatAsAtomicUnit=on  RTWFcnName=SUPPLIER_CALL_Fim_min_lpos1_4sl  mask(AEMS_SUPPLIER_CALL_FIM_MIN_LPOS1_4SL){}
      mask help:
      | Fuel injection minimum mass depending on rail pressure.
      |
      | This block is to call Supplier call API.
      mask init: same as AEMS_Standard_Library/SPECIFIC/AEMS_SUPPLIER_CALL_FIM_MIN_AFTR
      settings: AttributesFormatString=%<MaskType>  RTWSystemCode=Nonreusable function  RTWFcnNameOpts=User specified
      mask Help:
      | eval('path_lib=fileparts(which(''AEMS_Standard_Library''));');
      | mskblk=get_param(gcbh,'MaskType');
      | doc_path = [path_lib '\Help\',mskblk,'.pdf'];
      | eval('open(doc_path)');
  AEMS_SUPPLIER_CALL_FIM_MIN_LPOS2_2SL : Subsystem  Tag=[LIB]  TreatAsAtomicUnit=on  RTWFcnName=SUPPLIER_CALL_Fim_min_lpos2_2sl  mask(AEMS_SUPPLIER_CALL_FIM_MIN_LPOS2_2SL){}
      mask help:
      | Fuel injection minimum mass depending on rail pressure.
      |
      | This block is to call Supplier call API.
      mask init: same as AEMS_Standard_Library/SPECIFIC/AEMS_SUPPLIER_CALL_FIM_MIN_AFTR
      settings: AttributesFormatString=%<MaskType>  RTWSystemCode=Nonreusable function  RTWFcnNameOpts=User specified
      mask Help:
      | eval('path_lib=fileparts(which(''AEMS_Standard_Library''));');
      | mskblk=get_param(gcbh,'MaskType');
      | doc_path = [path_lib '\Help\',mskblk,'.pdf'];
      | eval('open(doc_path)');
  AEMS_SUPPLIER_CALL_FIM_MIN_LPOS2_3SL : Subsystem  Tag=[LIB]  TreatAsAtomicUnit=on  RTWFcnName=SUPPLIER_CALL_Fim_min_lpos2_3sl  mask(AEMS_SUPPLIER_CALL_FIM_MIN_LPOS2_3SL){}
      mask help:
      | Fuel injection minimum mass depending on rail pressure.
      |
      | This block is to call Supplier call API.
      mask init: same as AEMS_Standard_Library/SPECIFIC/AEMS_SUPPLIER_CALL_FIM_MIN_AFTR
      settings: AttributesFormatString=%<MaskType>  RTWSystemCode=Nonreusable function  RTWFcnNameOpts=User specified
      mask Help:
      | eval('path_lib=fileparts(which(''AEMS_Standard_Library''));');
      | mskblk=get_param(gcbh,'MaskType');
      | doc_path = [path_lib '\Help\',mskblk,'.pdf'];
      | eval('open(doc_path)');
  AEMS_SUPPLIER_CALL_FIM_MIN_LPOS2_4SL : Subsystem  Tag=[LIB]  TreatAsAtomicUnit=on  RTWFcnName=SUPPLIER_CALL_Fim_min_lpos2_4sl  mask(AEMS_SUPPLIER_CALL_FIM_MIN_LPOS2_4SL){}
      mask help:
      | Fuel injection minimum mass depending on rail pressure.
      |
      | This block is to call Supplier call API.
      mask init: same as AEMS_Standard_Library/SPECIFIC/AEMS_SUPPLIER_CALL_FIM_MIN_AFTR
      settings: AttributesFormatString=%<MaskType>  RTWSystemCode=Nonreusable function  RTWFcnNameOpts=User specified
      mask Help:
      | eval('path_lib=fileparts(which(''AEMS_Standard_Library''));');
      | mskblk=get_param(gcbh,'MaskType');
      | doc_path = [path_lib '\Help\',mskblk,'.pdf'];
      | eval('open(doc_path)');
  AEMS_SUPPLIER_CALL_FIM_MIN_LPOS3_3SL : Subsystem  Tag=[LIB]  TreatAsAtomicUnit=on  RTWFcnName=SUPPLIER_CALL_Fim_min_lpos3_3sl  mask(AEMS_SUPPLIER_CALL_FIM_MIN_LPOS3_3SL){}
      mask help:
      | Fuel injection minimum mass depending on rail pressure.
      |
      | This block is to call Supplier call API.
      mask init: same as AEMS_Standard_Library/SPECIFIC/AEMS_SUPPLIER_CALL_FIM_MIN_LPOS1
      settings: AttributesFormatString=%<MaskType>  RTWSystemCode=Nonreusable function  RTWFcnNameOpts=User specified
      mask Help:
      | eval('path_lib=fileparts(which(''AEMS_Standard_Library''));');
      | mskblk=get_param(gcbh,'MaskType');
      | doc_path = [path_lib '\Help\',mskblk,'.pdf'];
      | eval('open(doc_path)');
  AEMS_SUPPLIER_CALL_FIM_MIN_LPOS3_4SL : Subsystem  Tag=[LIB]  TreatAsAtomicUnit=on  RTWFcnName=SUPPLIER_CALL_Fim_min_lpos3_4sl  mask(AEMS_SUPPLIER_CALL_FIM_MIN_LPOS3_4SL){}
      mask help:
      | Fuel injection minimum mass depending on rail pressure.
      |
      | This block is to call Supplier call API.
      mask init: same as AEMS_Standard_Library/SPECIFIC/AEMS_SUPPLIER_CALL_FIM_MIN_LPOS1
      settings: AttributesFormatString=%<MaskType>  RTWSystemCode=Nonreusable function  RTWFcnNameOpts=User specified
      mask Help:
      | eval('path_lib=fileparts(which(''AEMS_Standard_Library''));');
      | mskblk=get_param(gcbh,'MaskType');
      | doc_path = [path_lib '\Help\',mskblk,'.pdf'];
      | eval('open(doc_path)');
  AEMS_SUPPLIER_CALL_FIM_MIN_LPOS4_4SL : Subsystem  Tag=[LIB]  TreatAsAtomicUnit=on  RTWFcnName=SUPPLIER_CALL_Fim_min_lpos4_4sl  mask(AEMS_SUPPLIER_CALL_FIM_MIN_LPOS4_4SL){}
      mask help:
      | Fuel injection minimum mass depending on rail pressure.
      |
      | This block is to call Supplier call API.
      mask init: same as AEMS_Standard_Library/SPECIFIC/AEMS_SUPPLIER_CALL_FIM_MIN_LPOS1
      settings: AttributesFormatString=%<MaskType>  RTWSystemCode=Nonreusable function  RTWFcnNameOpts=User specified
      mask Help:
      | eval('path_lib=fileparts(which(''AEMS_Standard_Library''));');
      | mskblk=get_param(gcbh,'MaskType');
      | doc_path = [path_lib '\Help\',mskblk,'.pdf'];
      | eval('open(doc_path)');
  AEMS_SUPPLIER_CALL_FIM_MIN_MAIN : Subsystem  Tag=[LIB]  TreatAsAtomicUnit=on  RTWFcnName=SUPPLIER_CALL_Fim_min_main  mask(AEMS_SUPPLIER_CALL_FIM_MIN_MAIN){}
      mask help:
      | Fuel injection minimum mass depending on rail pressure.
      |
      | This block is to call Supplier call API.
      mask init: same as AEMS_Standard_Library/SPECIFIC/AEMS_SUPPLIER_CALL_FIM_MIN_AFTR
      settings: AttributesFormatString=%<MaskType>  RTWSystemCode=Nonreusable function  RTWFcnNameOpts=User specified
      mask Help:
      | eval('path_lib=fileparts(which(''AEMS_Standard_Library''));');
      | mskblk=get_param(gcbh,'MaskType');
      | doc_path = [path_lib '\Help\',mskblk,'.pdf'];
      | eval('open(doc_path)');
  AEMS_SUPPLIER_CALL_FIM_MIN_PINJ1 : Subsystem  Tag=[LIB]  TreatAsAtomicUnit=on  RTWFcnName=SUPPLIER_CALL_Fim_min_pinj1  mask(AEMS_SUPPLIER_CALL_FIM_MIN_PINJ1){}
      mask help:
      | Fuel injection minimum mass depending on rail pressure.
      |
      | This block is to call Supplier call API.
      mask init: same as AEMS_Standard_Library/SPECIFIC/AEMS_SUPPLIER_CALL_FIM_MIN_AFTR
      settings: AttributesFormatString=%<MaskType>  RTWSystemCode=Nonreusable function  RTWFcnNameOpts=User specified
      mask Help:
      | eval('path_lib=fileparts(which(''AEMS_Standard_Library''));');
      | mskblk=get_param(gcbh,'MaskType');
      | doc_path = [path_lib '\Help\',mskblk,'.pdf'];
      | eval('open(doc_path)');
  AEMS_SUPPLIER_CALL_FIM_MIN_PINJ2 : Subsystem  Tag=[LIB]  TreatAsAtomicUnit=on  RTWFcnName=SUPPLIER_CALL_Fim_min_pinj2  mask(AEMS_SUPPLIER_CALL_FIM_MIN_PINJ2){}
      mask help:
      | Fuel injection minimum mass depending on rail pressure.
      |
      | This block is to call Supplier call API.
      mask init: same as AEMS_Standard_Library/SPECIFIC/AEMS_SUPPLIER_CALL_FIM_MIN_AFTR
      settings: AttributesFormatString=%<MaskType>  RTWSystemCode=Nonreusable function  RTWFcnNameOpts=User specified
      mask Help:
      | eval('path_lib=fileparts(which(''AEMS_Standard_Library''));');
      | mskblk=get_param(gcbh,'MaskType');
      | doc_path = [path_lib '\Help\',mskblk,'.pdf'];
      | eval('open(doc_path)');
  AEMS_SUPPLIER_CALL_FIM_MIN_PINJ3 : Subsystem  Tag=[LIB]  TreatAsAtomicUnit=on  RTWFcnName=SUPPLIER_CALL_Fim_min_pinj3  mask(AEMS_SUPPLIER_CALL_FIM_MIN_PINJ3){}
      mask help:
      | Fuel injection minimum mass depending on rail pressure.
      |
      | This block is to call Supplier call API.
      mask init: same as AEMS_Standard_Library/SPECIFIC/AEMS_SUPPLIER_CALL_FIM_MIN_AFTR
      settings: AttributesFormatString=%<MaskType>  RTWSystemCode=Nonreusable function  RTWFcnNameOpts=User specified
      mask Help:
      | eval('path_lib=fileparts(which(''AEMS_Standard_Library''));');
      | mskblk=get_param(gcbh,'MaskType');
      | doc_path = [path_lib '\Help\',mskblk,'.pdf'];
      | eval('open(doc_path)');
  AEMS_SUPPLIER_CALL_FIM_MIN_PINJ4 : Subsystem  Tag=[LIB]  TreatAsAtomicUnit=on  RTWFcnName=SUPPLIER_CALL_Fim_min_pinj4  mask(AEMS_SUPPLIER_CALL_FIM_MIN_PINJ4){}
      mask help:
      | Fuel injection minimum mass depending on rail pressure.
      |
      | This block is to call Supplier call API.
      mask init: same as AEMS_Standard_Library/SPECIFIC/AEMS_SUPPLIER_CALL_FIM_MIN_AFTR
      settings: AttributesFormatString=%<MaskType>  RTWSystemCode=Nonreusable function  RTWFcnNameOpts=User specified
      mask Help:
      | eval('path_lib=fileparts(which(''AEMS_Standard_Library''));');
      | mskblk=get_param(gcbh,'MaskType');
      | doc_path = [path_lib '\Help\',mskblk,'.pdf'];
      | eval('open(doc_path)');
  AEMS_SUPPLIER_CALL_FIM_MIN_POST : Subsystem  Tag=[LIB]  TreatAsAtomicUnit=on  RTWFcnName=SUPPLIER_CALL_Fim_min_post  mask(AEMS_SUPPLIER_CALL_FIM_MIN_POST){}
      mask help:
      | Fuel injection minimum mass depending on rail pressure.
      |
      | This block is to call Supplier call API.
      mask init: same as AEMS_Standard_Library/SPECIFIC/AEMS_SUPPLIER_CALL_FIM_MIN_AFTR
      settings: AttributesFormatString=%<MaskType>  RTWSystemCode=Nonreusable function  RTWFcnNameOpts=User specified
      mask Help:
      | eval('path_lib=fileparts(which(''AEMS_Standard_Library''));');
      | mskblk=get_param(gcbh,'MaskType');
      | doc_path = [path_lib '\Help\',mskblk,'.pdf'];
      | eval('open(doc_path)');
  AEMS_SUPPLIER_CALL_FUEL_INJ_MIN : Subsystem  Tag=[LIB]  TreatAsAtomicUnit=on  RTWFcnName=SUPPLIER_CALL_Fim_min_post1  mask(AEMS_SUPPLIER_CALL_FUEL_INJ_MIN){Outportname=Vxx_fms_fim_min_post1_3sl, Suppliercallname=SUPPLIER_CALL_Fim_min_post1, Splitnum=3}
      mask prompts: Outportname "Outport Name"; Suppliercallname "Supplier call Name"; Splitnum "Split"
      mask help:
      | Fuel injection minimum mass depending on rail pressure.
      |
      | Coding information: This block is to call Supplier call API.
      | Each block will be translated into code C by this way:
      | Output=Supplier call API Name(Splitnum);
      | Example for Supplier_Call_Fim_min_post1, corresponding output variable is
      | Vxx_fms_fim_min_post1= Supplier_Call_Fim_min_post1(1);
      mask init:
      | ThisBlk = gcb;
      | OutPorts            =   {'Vxx_fms_fim_min_post1','Vxx_fms_fim_min_post1_2sl','Vxx_fms_fim_min_post1_3sl','Vxx_fms_fim_min_post2_2sl','Vxx_fms_fim_min_post2_3sl','Vxx_fms_fim_min_post3_3sl'};
      | 
      | Supplier_Calls      =   {'SUPPLIER_CALL_Fim_min_post1','SUPPLIER_CALL_Fim_min_post1','SUPPLIER_CALL_Fim_min_post1','SUPPLIER_CALL_Fim_min_post2','SUPPLIER_CALL_Fim_min_post2','SUPPLIER_CALL_Fim_min_post3'};
      | 
      | Data_Names          =   {'Supplier_Call_Fim_min_post1','Supplier_Call_Fim_min_post1','Supplier_Call_Fim_min_post1','Supplier_Call_Fim_min_post2','Supplier_Call_Fim_min_post2','Supplier_Call_Fim_min_post3'};                     
      |                       
      |                       
      | Splits              =   {'1','2','3','2','3','3'};
      | 
      | model_type_pos = strsplit(ThisBlk,'/');
      | runnable_path = [bdroot '/' model_type_pos{2}];%to get the runnable or APICALL path
      | trg_port_name = get_param(find_system(runnable_path,'BlockType','TriggerPort'),'Name');%to get the function call trigger name
      | TaskRate = '';
      | if ~isempty(trg_port_name)
      |     trg_port_name_spltd = strsplit(trg_port_name{1},'_');
      |     if ~isempty(regexp(trg_port_name_spltd{1},'^Sched|^Event','once'))
      |         TaskRate = ['_' regexprep(trg_port_name_spltd{1},'Sched|Event','','once')];
      |     elseif ~isempty(regexp([trg_port_name_spltd{1} '_' trg_port_name_spltd{2} '_' ],'^DataServices_DCM_|^RoutineServices_DCM_','once'))||...
      |             ~isempty(regexp(trg_port_name_spltd{1},'^Dcm$','once'))
      |         TaskRate = '_dcmcb';
      |     elseif ~isempty(regexp(trg_port_name_spltd{1},'^Com$','once'))
      |         msg = sprintf(['\n','The Supplier call block "' Thisblk '" should not be present within APICALLs having function call trigger as "Com"']);
      |         errordlg(msg);
      |         return;
      |     end
      | end
      | 
      | Idx_Of_Outportname = find(ismember(OutPorts,Outportname));
      | DataName = [Data_Names{Idx_Of_Outportname} TaskRate];
      | 
      | %set the  suppliername according to the Outport name.
      | set_param(ThisBlk,'Suppliercallname',Supplier_Calls{Idx_Of_Outportname});
      | set_param(ThisBlk,'Splitnum',Splits{Idx_Of_Outportname});
      | 
      | %Get the paths of the blks under this lib block.
      | Const_Blk = [ThisBlk,'/Splitnum'];%%path of "const block" inside this lib blk.
      | DSR_Blk   = [ThisBlk,'/Data_Store_Read'];%path of "Data store read block" inside this lib blk.
      | Outport_Blk = find_system(ThisBlk,'LookUnderMasks','all','FollowLinks','on','BlockType','Outport');
      | Outport_Blk = Outport_Blk{1};%I know this is d only outport blk.
      | 
      | %set the attributes of the blks under this lib block, based on teh Outportname chosen by d user.
      | set_param(Outport_Blk,'Name',Outportname);
      | set_param(DSR_Blk,'DataStoreName',DataName);
      | set_param(Const_Blk,'Value',Splits{Idx_Of_Outportname});
      | 
      | %To create a singal object in d base workspace.
      | EvalStr = ['exist(''',DataName,''',''var'')'];
      | structVxx=Simulink.Signal;
      | % structVxx=Simulink.Signal;
      | structVxx.Dimensions=1;
      | structVxx.DimensionsMode='Fixed';
      | structVxx.DataType='single';
      | structVxx.Complexity='real';
      | structVxx.SamplingMode='Sample based';
      | structVxx.SampleTime=-1;
      | isDefined= evalin('base',EvalStr);%This line checks whether the DataName exist in the base workspace.
      | if (isDefined==0)
      |     assignin('base',DataName,structVxx);
      | end
      settings: RTWSystemCode=Inline  RTWFcnNameOpts=User specified
      settings: AttributesFormatString=|
      | %<MaskType>
      | Supplier Call Name = %<Suppliercallname>
      | Outport Name = %<Outportname>\nSplit Number= %<Splitnum>
      mask Help:
      | eval('path_lib=fileparts(which(''AEMS_Standard_Library''));');
      | mskblk=get_param(gcbh,'MaskType');
      | doc_path = [path_lib '\Help\',mskblk,'.pdf'];
      | eval('open(doc_path)');
      mask TypeOptions Outportname: Vxx_fms_fim_min_post1 | Vxx_fms_fim_min_post1_2sl | Vxx_fms_fim_min_post1_3sl | Vxx_fms_fim_min_post2_2sl | Vxx_fms_fim_min_post2_3sl | Vxx_fms_fim_min_post3_3sl
      mask Callback Outportname:
      | OutPorts            =   {'Vxx_fms_fim_min_post1','Vxx_fms_fim_min_post1_2sl','Vxx_fms_fim_min_post1_3sl','Vxx_fms_fim_min_post2_2sl','Vxx_fms_fim_min_post2_3sl','Vxx_fms_fim_min_post3_3sl'};
      | 
      | Supplier_Calls      =   {'SUPPLIER_CALL_Fim_min_post1','SUPPLIER_CALL_Fim_min_post1','SUPPLIER_CALL_Fim_min_post1','SUPPLIER_CALL_Fim_min_post2','SUPPLIER_CALL_Fim_min_post2','SUPPLIER_CALL_Fim_min_post3'};
      | 
      | Splits              =   {'1','2','3','2','3','3'};
      | 
      | Outportname = get_param(gcb,'Outportname');
      | 
      | Idx_Of_Outportname = find(ismember(OutPorts,Outportname));
      | %set the  suppliername according to the Outport name.
      | set_param(gcb,'Suppliercallname',Supplier_Calls{Idx_Of_Outportname});
      | set_param(gcb,'Splitnum',Splits{Idx_Of_Outportname});
      | cellfun(@clear,{'Idx_Of_Outportname','Outportname','OutPorts','Splits','Supplier_Calls'});
  AEMS_SUPPLIER_CALL_ICLC_LEARNING : Subsystem  Tag=[LIB]  TreatAsAtomicUnit=on  RTWFcnName=SUPPLIER_CALL_Esti_ti_aftr  mask(AEMS_SUPPLIER_CALL_ICLC_LEARNING){}
      mask help: Supplier Call Block for ICLC_LEARNING
      mask init:
      | Thisblk = gcb;
      | model_type_pos = strsplit(Thisblk,'/');%to split all the layer paths in order to get the runnable path
      | runnable_path = [bdroot '/' model_type_pos{2}];%to get the runnable or AIPCALL path
      | trg_port_name = get_param(find_system(runnable_path,'BlockType','TriggerPort'),'Name');%to get the function call trigger name
      | TaskRate = '';%the raster suffix is stored in the parameter 
      | 
      | if ~isempty(trg_port_name)
      |     trg_port_name_spltd = strsplit(trg_port_name{1},'_');%splitting is done in order to get the raster and its type(Sched or Event)
      |     
      |     % checking for rasters of type Sched or Event especially occuring in
      |     % runnables
      |     if ~isempty(regexp(trg_port_name_spltd{1},'^Sched|^Event','once')) 
      |         TaskRate = ['_' regexprep(trg_port_name_spltd{1},'Sched|Event','','once')];
      |         
      |     %checking if the raster is dcmcb and this is applicable only for
      |     %APICALL
      |     elseif ~isempty(regexp([trg_port_name_spltd{1} '_' trg_port_name_spltd{2} '_' ],'^DataServices_DCM_|^RoutineServices_DCM_','once'))||...
      |             ~isempty(regexp(trg_port_name_spltd{1},'^Dcm$','once'))
      |         TaskRate = '_dcmcb';
      |         
      |     %checking if this block is used under the function call trigger
      |     %starting with "Com" and then giving an error message
      |     %this is applicable only for APICALL
      |     elseif ~isempty(regexp(trg_port_name_spltd{1},'^Com$','once'))
      |         msg = sprintf(['\n','The Supplier call block "' Thisblk '" should not be present within APICALLs having function call trigger as "Com"']);
      |         errordlg(msg);
      |         return;
      |     end
      | end
      | 
      | DataName = ['Supplier_call_ICLC_learning_request' TaskRate];%the variable name that should be given to DataStoreRead block 
      | DataName1 = ['Supplier_call_ICLC_learning_MFF_1' TaskRate];
      | set_param([Thisblk '/DataStoreRead'],'DataStoreName',DataName);%Setting the DataStoreName of DataStoreRead block
      | set_param([Thisblk '/DataStoreRead1'],'DataStoreName',DataName1);%Setting the DataStoreName of DataStoreRead1 block
      | 
      | %other settings done to this variable name
      | structVbx=Simulink.Signal;
      | structVbx.Dimensions=1;
      | structVbx.DimensionsMode='Fixed';
      | structVbx.DataType='boolean';
      | structVbx.Complexity='real';
      | structVbx.SamplingMode='Sample based';
      | structVbx.SampleTime=-1;
      | assignin('base',DataName,structVbx); 
      | 
      | %other settings done to this variable name
      | structVxx=Simulink.Signal;
      | structVxx.Dimensions=1;
      | structVxx.DimensionsMode='Fixed';
      | structVxx.DataType='single';
      | structVxx.Complexity='real';
      | structVxx.SamplingMode='Sample based';
      | structVxx.SampleTime=-1;
      | assignin('base',DataName1,structVxx);
      settings: AttributesFormatString=%<MaskType>  RTWSystemCode=Nonreusable function  RTWFcnNameOpts=User specified
      mask Help:
      | eval('path_lib=fileparts(which(''AEMS_Standard_Library''));');
      | doc_path = [path_lib '\help\AEMS_SUPPLIER_CALL_ICLC_LEARNING.pdf'];
      | eval('open(doc_path)')
  AEMS_SUPPLIER_CALL_MAX_NBR_INJ : Subsystem  Tag=[LIB]  TreatAsAtomicUnit=on  RTWFcnName=SUPPLIER_CALL_Max_nbr_inj  mask(AEMS_SUPPLIER_CALL_MAX_NBR_INJ){}
      mask help:
      | maximum number of injection available by the system,
      | 	depending on the engine speed
      | 	depending on the voltage battery
      |
      | This block is to call Supplier call API.
      mask init:
      | Thisblk = gcb;
      | model_type_pos = strsplit(Thisblk,'/');%to split all the layer paths in order to get the runnable path
      | runnable_path = [bdroot '/' model_type_pos{2}];%to get the runnable or AIPCALL path
      | trg_port_name = get_param(find_system(runnable_path,'BlockType','TriggerPort'),'Name');%to get the function call trigger name
      | TaskRate = '';%the raster suffix is stored in the parameter 
      | 
      | if ~isempty(trg_port_name)
      |     trg_port_name_spltd = strsplit(trg_port_name{1},'_');%splitting is done in order to get the raster and its type(Sched or Event)
      |     
      |     % checking for rasters of type Sched or Event especially occuring in
      |     % runnables
      |     if ~isempty(regexp(trg_port_name_spltd{1},'^Sched|^Event','once')) 
      |         TaskRate = ['_' regexprep(trg_port_name_spltd{1},'Sched|Event','','once')];
      |         
      |     %checking if the raster is dcmcb and this is applicable only for
      |     %APICALL
      |     elseif ~isempty(regexp([trg_port_name_spltd{1} '_' trg_port_name_spltd{2} '_' ],'^DataServices_DCM_|^RoutineServices_DCM_','once'))||...
      |             ~isempty(regexp(trg_port_name_spltd{1},'^Dcm$','once'))
      |         TaskRate = '_dcmcb';
      |         
      |     %checking if this block is used under the function call trigger
      |     %starting with "Com" and then giving an error message
      |     %this is applicable only for APICALL
      |     elseif ~isempty(regexp(trg_port_name_spltd{1},'^Com$','once'))
      |         msg = sprintf(['\n','The Supplier call block "' Thisblk '" should not be present within APICALLs having function call trigger as "Com"']);
      |         errordlg(msg);
      |         return;
      |     end
      | end
      | 
      | DataName = ['Supplier_call_nbr_inj_max' TaskRate];%the variable name that should be given to DataStoreRead block 
      | set_param([Thisblk '/Data Store Read'],'DataStoreName',DataName);%Setting the DataStoreName of DataStoreRead block
      | 
      | %other settings done to this variable name
      | structVxx=Simulink.Signal;
      | structVxx.Dimensions=1;
      | structVxx.DimensionsMode='Fixed';
      | structVxx.DataType='uint8';
      | structVxx.Complexity='real';
      | structVxx.SamplingMode='Sample based';
      | structVxx.SampleTime=-1;
      | assignin('base',DataName,structVxx);
      settings: AttributesFormatString=%<MaskType>  RTWSystemCode=Nonreusable function  RTWFcnNameOpts=User specified
      mask Help:
      | eval('path_lib=fileparts(which(''AEMS_Standard_Library''));');
      | mskblk=get_param(gcbh,'MaskType');
      | doc_path = [path_lib '\Help\',mskblk,'.pdf'];
      | eval('open(doc_path)');
  AEMS_SUPPLIER_CALL_PHI_MAX_PINJ1 : Subsystem  Tag=[LIB]  TreatAsAtomicUnit=on  RTWFcnName=SUPPLIER_CALL_Phi_max_pinj1  mask(AEMS_SUPPLIER_CALL_PHI_MAX_PINJ1){}
      mask help: Maximal angle where the last injection has to be finished.
      mask init:
      | Thisblk = gcb;
      | model_type_pos = strsplit(Thisblk,'/');%to split all the layer paths in order to get the runnable path
      | runnable_path = [bdroot '/' model_type_pos{2}];%to get the runnable or AIPCALL path
      | trg_port_name = get_param(find_system(runnable_path,'BlockType','TriggerPort'),'Name');%to get the function call trigger name
      | TaskRate = '';%the raster suffix is stored in the parameter 
      | 
      | if ~isempty(trg_port_name)
      |     trg_port_name_spltd = strsplit(trg_port_name{1},'_');%splitting is done in order to get the raster and its type(Sched or Event)
      |     
      |     % checking for rasters of type Sched or Event especially occuring in
      |     % runnables
      |     if ~isempty(regexp(trg_port_name_spltd{1},'^Sched|^Event','once')) 
      |         TaskRate = ['_' regexprep(trg_port_name_spltd{1},'Sched|Event','','once')];
      |         
      |     %checking if the raster is dcmcb and this is applicable only for
      |     %APICALL
      |     elseif ~isempty(regexp([trg_port_name_spltd{1} '_' trg_port_name_spltd{2} '_' ],'^DataServices_DCM_|^RoutineServices_DCM_','once'))||...
      |             ~isempty(regexp(trg_port_name_spltd{1},'^Dcm$','once'))
      |         TaskRate = '_dcmcb';
      |         
      |     %checking if this block is used under the function call trigger
      |     %starting with "Com" and then giving an error message
      |     %this is applicable only for APICALL
      |     elseif ~isempty(regexp(trg_port_name_spltd{1},'^Com$','once'))
      |         msg = sprintf(['\n','The Supplier call block "' Thisblk '" should not be present within APICALLs having function call trigger as "Com"']);
      |         errordlg(msg);
      |         return;
      |     end
      | end
      | 
      | DataName = ['Supplier_Call_Phi_Max' TaskRate];%the variable name that should be given to DataStoreRead block 
      | set_param([Thisblk '/Data Store Read'],'DataStoreName',DataName);%Setting the DataStoreName of DataStoreRead block
      | 
      | %other settings done to this variable name
      | structVxx=Simulink.Signal;
      | structVxx.Dimensions=1;
      | structVxx.DimensionsMode='Fixed';
      | structVxx.DataType='single';
      | structVxx.Complexity='real';
      | structVxx.SamplingMode='Sample based';
      | structVxx.SampleTime=-1;
      | assignin('base',DataName,structVxx);
      settings: AttributesFormatString=%<MaskType>  RTWSystemCode=Nonreusable function  RTWFcnNameOpts=User specified
      mask Help:
      | eval('path_lib=fileparts(which(''AEMS_Standard_Library''));');
      | mskblk=get_param(gcbh,'MaskType');
      | doc_path = [path_lib '\Help\',mskblk,'.pdf'];
      | eval('open(doc_path)');
  AEMS_SUPPLIER_CALL_PHI_MAX_PINJ2 : Subsystem  Tag=[LIB]  TreatAsAtomicUnit=on  RTWFcnName=SUPPLIER_CALL_Phi_max_pinj2  mask(AEMS_SUPPLIER_CALL_PHI_MAX_PINJ2){}
      mask help: Maximal angle where the last injection has to be finished.
      mask init: same as AEMS_Standard_Library/SPECIFIC/AEMS_SUPPLIER_CALL_PHI_MAX_PINJ1
      settings: AttributesFormatString=%<MaskType>  RTWSystemCode=Nonreusable function  RTWFcnNameOpts=User specified
      mask Help:
      | eval('path_lib=fileparts(which(''AEMS_Standard_Library''));');
      | mskblk=get_param(gcbh,'MaskType');
      | doc_path = [path_lib '\Help\',mskblk,'.pdf'];
      | eval('open(doc_path)');
  AEMS_SUPPLIER_CALL_PHI_MAX_PINJ3 : Subsystem  Tag=[LIB]  TreatAsAtomicUnit=on  RTWFcnName=SUPPLIER_CALL_Phi_max_pinj3  mask(AEMS_SUPPLIER_CALL_PHI_MAX_PINJ3){}
      mask help: Maximal angle where the last injection has to be finished.
      mask init: same as AEMS_Standard_Library/SPECIFIC/AEMS_SUPPLIER_CALL_PHI_MAX_PINJ1
      settings: AttributesFormatString=%<MaskType>  RTWSystemCode=Nonreusable function  RTWFcnNameOpts=User specified
      mask Help:
      | eval('path_lib=fileparts(which(''AEMS_Standard_Library''));');
      | mskblk=get_param(gcbh,'MaskType');
      | doc_path = [path_lib '\Help\',mskblk,'.pdf'];
      | eval('open(doc_path)');
  AEMS_SUPPLIER_CALL_PHI_MAX_PINJ4 : Subsystem  Tag=[LIB]  TreatAsAtomicUnit=on  RTWFcnName=SUPPLIER_CALL_Phi_max_pinj4  mask(AEMS_SUPPLIER_CALL_PHI_MAX_PINJ4){}
      mask help: Maximal angle where the last injection has to be finished.
      mask init: same as AEMS_Standard_Library/SPECIFIC/AEMS_SUPPLIER_CALL_PHI_MAX_PINJ1
      settings: AttributesFormatString=%<MaskType>  RTWSystemCode=Nonreusable function  RTWFcnNameOpts=User specified
      mask Help:
      | eval('path_lib=fileparts(which(''AEMS_Standard_Library''));');
      | mskblk=get_param(gcbh,'MaskType');
      | doc_path = [path_lib '\Help\',mskblk,'.pdf'];
      | eval('open(doc_path)');
  AEMS_SUPPLIER_CALL_PHI_MIN_AFTR : Subsystem  Tag=[LIB]  TreatAsAtomicUnit=on  RTWFcnName=SUPPLIER_CALL_Phi_min_aftr  mask(AEMS_SUPPLIER_CALL_PHI_MIN_AFTR){}
      mask help: SUPPLIER_CALL_phi_min
      mask init:
      | Thisblk = gcb;
      | model_type_pos = strsplit(Thisblk,'/');%to split all the layer paths in order to get the runnable path
      | runnable_path = [bdroot '/' model_type_pos{2}];%to get the runnable or AIPCALL path
      | trg_port_name = get_param(find_system(runnable_path,'BlockType','TriggerPort'),'Name');%to get the function call trigger name
      | TaskRate = '';%the raster suffix is stored in the parameter 
      | 
      | if ~isempty(trg_port_name)
      |     trg_port_name_spltd = strsplit(trg_port_name{1},'_');%splitting is done in order to get the raster and its type(Sched or Event)
      |     
      |     % checking for rasters of type Sched or Event especially occuring in
      |     % runnables
      |     if ~isempty(regexp(trg_port_name_spltd{1},'^Sched|^Event','once')) 
      |         TaskRate = ['_' regexprep(trg_port_name_spltd{1},'Sched|Event','','once')];
      |         
      |     %checking if the raster is dcmcb and this is applicable only for
      |     %APICALL
      |     elseif ~isempty(regexp([trg_port_name_spltd{1} '_' trg_port_name_spltd{2} '_' ],'^DataServices_DCM_|^RoutineServices_DCM_','once'))||...
      |             ~isempty(regexp(trg_port_name_spltd{1},'^Dcm$','once'))
      |         TaskRate = '_dcmcb';
      |         
      |     %checking if this block is used under the function call trigger
      |     %starting with "Com" and then giving an error message
      |     %this is applicable only for APICALL
      |     elseif ~isempty(regexp(trg_port_name_spltd{1},'^Com$','once'))
      |         msg = sprintf(['\n','The Supplier call block "' Thisblk '" should not be present within APICALLs having function call trigger as "Com"']);
      |         errordlg(msg);
      |         return;
      |     end
      | end
      | 
      | DataName = ['Supplier_Call_Phi_Min' TaskRate];%the variable name that should be given to DataStoreRead block 
      | set_param([Thisblk '/Data Store Read'],'DataStoreName',DataName);%Setting the DataStoreName of DataStoreRead block
      | 
      | %other settings done to this variable name
      | structVxx=Simulink.Signal;
      | structVxx.Dimensions=1;
      | structVxx.DimensionsMode='Fixed';
      | structVxx.DataType='single';
      | structVxx.Complexity='real';
      | structVxx.SamplingMode='Sample based';
      | structVxx.SampleTime=-1;
      | assignin('base',DataName,structVxx);
      settings: AttributesFormatString=%<MaskType>  RTWSystemCode=Nonreusable function  RTWFcnNameOpts=User specified
      mask Help:
      | eval('path_lib=fileparts(which(''AEMS_Standard_Library''));');
      | mskblk=get_param(gcbh,'MaskType');
      | doc_path = [path_lib '\Help\',mskblk,'.pdf'];
      | eval('open(doc_path)');
  AEMS_SUPPLIER_CALL_PHI_MIN_ING : Subsystem  Tag=[LIB]  TreatAsAtomicUnit=on  RTWFcnName=SUPPLIER_CALL_Phi_min_post1  mask(AEMS_SUPPLIER_CALL_PHI_MIN_ING){Outportname=Vxx_fms_phi_min_post3, Suppliercallname=SUPPLIER_CALL_Phi_min_post3}
      mask prompts: Outportname "Outport Name"; Suppliercallname "Supplier call Name"
      mask help:
      | Minimal angle where the last injection has to be finished.
      |
      | Each block will be translated into code C by this way:
      | Output=Supplier call API Name
      | Example for Supplier_Call_Phi_min_post1, corresponding output variable is Vxx_fms_phi_min_post1
      | Vxx_fms_phi_min_post1= Supplier_Call_Phi_min_post1
      mask init:
      | ThisBlk = gcb;
      | OutPorts            =   {'Vxx_fms_phi_min_post1','Vxx_fms_phi_min_post2','Vxx_fms_phi_min_post3'};
      | 
      | Supplier_Calls      =   {'SUPPLIER_CALL_Phi_min_post1','SUPPLIER_CALL_Phi_min_post2','SUPPLIER_CALL_Phi_min_post3'};
      | 
      | Data_Names         =    {'Supplier_Call_Phi_min_post1','Supplier_Call_Phi_min_post2','Supplier_Call_Phi_min_post3'};
      | 
      | model_type_pos = strsplit(ThisBlk,'/');
      | runnable_path = [bdroot '/' model_type_pos{2}];%to get the runnable or APICALL path
      | trg_port_name = get_param(find_system(runnable_path,'BlockType','TriggerPort'),'Name');%to get the function call trigger name
      | TaskRate = '';
      | if ~isempty(trg_port_name)
      |     trg_port_name_spltd = strsplit(trg_port_name{1},'_');
      |     if ~isempty(regexp(trg_port_name_spltd{1},'^Sched|^Event','once'))
      |         TaskRate = ['_' regexprep(trg_port_name_spltd{1},'Sched|Event','','once')];
      |     elseif ~isempty(regexp([trg_port_name_spltd{1} '_' trg_port_name_spltd{2} '_' ],'^DataServices_DCM_|^RoutineServices_DCM_','once'))||...
      |             ~isempty(regexp(trg_port_name_spltd{1},'^Dcm$','once'))
      |         TaskRate = '_dcmcb';
      |     elseif ~isempty(regexp(trg_port_name_spltd{1},'^Com$','once'))
      |         msg = sprintf(['\n','The Supplier call block "' Thisblk '" should not be present within APICALLs having function call trigger as "Com"']);
      |         errordlg(msg);
      |         return;
      |     end
      | end
      | 
      | Idx_Of_Outportname = find(ismember(OutPorts,Outportname));
      | DataName = [Data_Names{Idx_Of_Outportname} TaskRate];
      | 
      | %set the  suppliername according to the Outport name.
      | set_param(ThisBlk,'Suppliercallname',Supplier_Calls{Idx_Of_Outportname});
      | 
      | %Get the paths of the blks under this lib block.
      | DSR_Blk   = [ThisBlk,'/Data_Store_Read'];%path of "Data store read block" inside this lib blk.
      | Outport_Blk = find_system(ThisBlk,'LookUnderMasks','all','FollowLinks','on','BlockType','Outport');
      | Outport_Blk = Outport_Blk{1};%I know this is d only outport blk.
      | 
      | %set the attributes of the blks under this lib block, based on teh Outportname chosen by d user.
      | set_param(Outport_Blk,'Name',Outportname);
      | set_param(DSR_Blk,'DataStoreName',DataName);
      | 
      | %To create a singal object in d base workspace.
      | EvalStr = ['exist(''',DataName,''',''var'')'];
      | structVxx=Simulink.Signal;
      | % structVxx=Simulink.Signal;
      | structVxx.Dimensions=1;
      | structVxx.DimensionsMode='Fixed';
      | structVxx.DataType='single';
      | structVxx.Complexity='real';
      | structVxx.SamplingMode='Sample based';
      | structVxx.SampleTime=-1;
      | isDefined= evalin('base',EvalStr);%This line checks whether the DataName exist in the base workspace.
      | if (isDefined==0)
      |     assignin('base',DataName,structVxx);
      | end
      settings: RTWSystemCode=Inline  RTWFcnNameOpts=User specified
      settings: AttributesFormatString=|
      | %<MaskType>
      | Outport Name = %<Outportname>
      | Supplier Call Name = %<Suppliercallname>
      mask Help:
      | eval('path_lib=fileparts(which(''AEMS_Standard_Library''));');
      | mskblk=get_param(gcbh,'MaskType');
      | doc_path = [path_lib '\Help\',mskblk,'.pdf'];
      | eval('open(doc_path)');
      mask TypeOptions Outportname: Vxx_fms_phi_min_post1 | Vxx_fms_phi_min_post2 | Vxx_fms_phi_min_post3
      mask Callback Outportname:
      | OutPorts            =   {'Vxx_fms_phi_min_post1','Vxx_fms_phi_min_post2','Vxx_fms_phi_min_post3'};
      | 
      | Supplier_Calls      =   {'SUPPLIER_CALL_Phi_min_post1','SUPPLIER_CALL_Phi_min_post2','SUPPLIER_CALL_Phi_min_post3'};
      | 
      | Data_Names         =    {'Supplier_Call_Phi_min_post1','Supplier_Call_Phi_min_post2','Supplier_Call_Phi_min_post3'};
      | 
      | 
      | Outportname = get_param(gcb,'Outportname');
      | 
      | Idx_Of_Outportname = find(ismember(OutPorts,Outportname));
      | %set the  suppliername according to the Outport name.
      | set_param(gcb,'Suppliercallname',Supplier_Calls{Idx_Of_Outportname});
      | cellfun(@clear,{'Idx_Of_Outportname','Outportname','OutPorts','Supplier_Calls','Data_Names'});
  AEMS_SUPPLIER_CALL_PHI_MIN_LPOS : Subsystem  Tag=[LIB]  TreatAsAtomicUnit=on  RTWFcnName=SUPPLIER_CALL_Phi_min_lpos  mask(AEMS_SUPPLIER_CALL_PHI_MIN_LPOS){}
      mask help: Minimal angle where the last injection has to be finished.
      mask init: same as AEMS_Standard_Library/SPECIFIC/AEMS_SUPPLIER_CALL_PHI_MIN_AFTR
      settings: AttributesFormatString=%<MaskType>  RTWSystemCode=Nonreusable function  RTWFcnNameOpts=User specified
      mask Help:
      | eval('path_lib=fileparts(which(''AEMS_Standard_Library''));');
      | mskblk=get_param(gcbh,'MaskType');
      | doc_path = [path_lib '\Help\',mskblk,'.pdf'];
      | eval('open(doc_path)');
  AEMS_SUPPLIER_CALL_PHI_MIN_LPOS2 : Subsystem  Tag=[LIB]  TreatAsAtomicUnit=on  RTWFcnName=SUPPLIER_CALL_Phi_min_lpos2  mask(AEMS_SUPPLIER_CALL_PHI_MIN_LPOS2){}
      mask help: Minimal angle where the last injection has to be finished.
      mask init: same as AEMS_Standard_Library/SPECIFIC/AEMS_SUPPLIER_CALL_PHI_MIN_AFTR
      settings: AttributesFormatString=%<MaskType>  RTWSystemCode=Nonreusable function  RTWFcnNameOpts=User specified
      mask Help:
      | eval('path_lib=fileparts(which(''AEMS_Standard_Library''));');
      | mskblk=get_param(gcbh,'MaskType');
      | doc_path = [path_lib '\Help\',mskblk,'.pdf'];
      | eval('open(doc_path)');
  AEMS_SUPPLIER_CALL_PHI_MIN_LPOS3 : Subsystem  Tag=[LIB]  TreatAsAtomicUnit=on  RTWFcnName=SUPPLIER_CALL_Phi_min_lpos3  mask(AEMS_SUPPLIER_CALL_PHI_MIN_LPOS3){}
      mask help: Minimal angle where the last injection has to be finished.
      mask init: same as AEMS_Standard_Library/SPECIFIC/AEMS_SUPPLIER_CALL_PHI_MIN_AFTR
      settings: AttributesFormatString=%<MaskType>  RTWSystemCode=Nonreusable function  RTWFcnNameOpts=User specified
      mask Help:
      | eval('path_lib=fileparts(which(''AEMS_Standard_Library''));');
      | mskblk=get_param(gcbh,'MaskType');
      | doc_path = [path_lib '\Help\',mskblk,'.pdf'];
      | eval('open(doc_path)');
  AEMS_SUPPLIER_CALL_PHI_MIN_LPOS4 : Subsystem  Tag=[LIB]  TreatAsAtomicUnit=on  RTWFcnName=SUPPLIER_CALL_Phi_min_lpos4  mask(AEMS_SUPPLIER_CALL_PHI_MIN_LPOS4){}
      mask help: Minimal angle where the last injection has to be finished.
      mask init: same as AEMS_Standard_Library/SPECIFIC/AEMS_SUPPLIER_CALL_PHI_MIN_AFTR
      settings: AttributesFormatString=%<MaskType>  RTWSystemCode=Nonreusable function  RTWFcnNameOpts=User specified
      mask Help:
      | eval('path_lib=fileparts(which(''AEMS_Standard_Library''));');
      | mskblk=get_param(gcbh,'MaskType');
      | doc_path = [path_lib '\Help\',mskblk,'.pdf'];
      | eval('open(doc_path)');
  AEMS_SUPPLIER_CALL_PHI_MIN_POST : Subsystem  Tag=[LIB]  TreatAsAtomicUnit=on  RTWFcnName=SUPPLIER_CALL_Phi_min_post  mask(AEMS_SUPPLIER_CALL_PHI_MIN_POST){}
      mask help: Minimal angle where the last injection has to be finished.
      mask init: same as AEMS_Standard_Library/SPECIFIC/AEMS_SUPPLIER_CALL_PHI_MIN_AFTR
      settings: AttributesFormatString=%<MaskType>  RTWSystemCode=Nonreusable function  RTWFcnNameOpts=User specified
      mask Help:
      | eval('path_lib=fileparts(which(''AEMS_Standard_Library''));');
      | mskblk=get_param(gcbh,'MaskType');
      | doc_path = [path_lib '\Help\',mskblk,'.pdf'];
      | eval('open(doc_path)');
  AEMS_SUPPLIER_CALL_QBA_TQI_MAX_LIM : Subsystem  Tag=[LIB]  TreatAsAtomicUnit=on  RTWFcnName=SUPPLIER_CALL_QBA_TQI_MAX_LIM  mask(AEMS_SUPPLIER_CALL_QBA_TQI_MAX_LIM){Suppliercallname=SUPPLIER_CALL_QBA_TQI_MAX_LIM}
      mask prompts: Suppliercallname "Supplier Call Name"
      mask help:
      | Get maximum torque due to QBA limitation from indicated torque raw without QBA limitation and set point via Supplier call function.
      |
      | -INPUTS-
      | Tqi_raw_wio_qba: indicated torque raw without QBA limitation
      | Tqi_sp: indicated torque set point
      |
      | -OUTPUTS-
      | Tqi_max_lim_qba: Maximum torque due to QBA limitation
      mask init:
      | Thisblk = gcb;
      | model_type_pos = strsplit(Thisblk,'/');%to split all the layer paths in order to get the runnable path
      | runnable_path = [bdroot '/' model_type_pos{2}];%to get the runnable or AIPCALL path
      | trg_port_name = get_param(find_system(runnable_path,'BlockType','TriggerPort'),'Name');%to get the function call trigger name
      | TaskRate = '';%the raster suffix is stored in the parameter 
      | 
      | if ~isempty(trg_port_name)
      |     trg_port_name_spltd = strsplit(trg_port_name{1},'_');%splitting is done in order to get the raster and its type(Sched or Event)
      |     
      |     % checking for rasters of type Sched or Event especially occuring in
      |     % runnables
      |     if ~isempty(regexp(trg_port_name_spltd{1},'^Sched|^Event','once')) 
      |         TaskRate = ['_' regexprep(trg_port_name_spltd{1},'Sched|Event','','once')];
      |         
      |     %checking if the raster is dcmcb and this is applicable only for
      |     %APICALL
      |     elseif ~isempty(regexp([trg_port_name_spltd{1} '_' trg_port_name_spltd{2} '_' ],'^DataServices_DCM_|^RoutineServices_DCM_','once'))||...
      |             ~isempty(regexp(trg_port_name_spltd{1},'^Dcm$','once'))
      |         TaskRate = '_dcmcb';
      |         
      |     %checking if this block is used under the function call trigger
      |     %starting with "Com" and then giving an error message
      |     %this is applicable only for APICALL
      |     elseif ~isempty(regexp(trg_port_name_spltd{1},'^Com$','once'))
      |         msg = sprintf(['\n','The Supplier call block "' Thisblk '" should not be present within APICALLs having function call trigger as "Com"']);
      |         errordlg(msg);
      |         return;
      |     end
      | end
      | 
      | DataName = ['Supplier_Call_QBA_TQI_MAX_LIM' TaskRate];%the variable name that should be given to DataStoreRead block 
      | set_param([Thisblk '/Supplier_Call_QBA_TQI_MAX_LIM'],'DataStoreName',DataName);%Setting the DataStoreName of DataStoreRead block
      | 
      | %other settings done to this variable name
      | structVxx=Simulink.Signal;
      | structVxx.Dimensions=1;
      | structVxx.DimensionsMode='Fixed';
      | structVxx.DataType='single';
      | structVxx.Complexity='real';
      | structVxx.SamplingMode='Sample based';
      | structVxx.SampleTime=-1;
      | assignin('base',DataName,structVxx);
      settings: RTWSystemCode=Inline  RTWFcnNameOpts=User specified
      settings: AttributesFormatString=|
      | %<MaskType>
      | Supplier Call Name = %<Suppliercallname>
      mask Help:
      | eval('path_lib=fileparts(which(''AEMS_Standard_Library''));');
      | mskblk=get_param(gcbh,'MaskType');
      | doc_path = [path_lib '\Help\',mskblk,'.pdf'];
      | eval('open(doc_path)');
  AEMS_SUPPLIER_CALL_SEPA_MIN_AFTR : Subsystem  Tag=[LIB]  TreatAsAtomicUnit=on  RTWFcnName=SUPPLIER_CALL_Sepa_min_aftr  mask(AEMS_SUPPLIER_CALL_SEPA_MIN_AFTR){}
      mask help: SUPPLIER_CALL_Sepa_min
      mask init:
      | Thisblk = gcb;
      | model_type_pos = strsplit(Thisblk,'/');%to split all the layer paths in order to get the runnable path
      | runnable_path = [bdroot '/' model_type_pos{2}];%to get the runnable or AIPCALL path
      | trg_port_name = get_param(find_system(runnable_path,'BlockType','TriggerPort'),'Name');%to get the function call trigger name
      | TaskRate = '';%the raster suffix is stored in the parameter 
      | 
      | if ~isempty(trg_port_name)
      |     trg_port_name_spltd = strsplit(trg_port_name{1},'_');%splitting is done in order to get the raster and its type(Sched or Event)
      |     
      |     % checking for rasters of type Sched or Event especially occuring in
      |     % runnables
      |     if ~isempty(regexp(trg_port_name_spltd{1},'^Sched|^Event','once')) 
      |         TaskRate = ['_' regexprep(trg_port_name_spltd{1},'Sched|Event','','once')];
      |         
      |     %checking if the raster is dcmcb and this is applicable only for
      |     %APICALL
      |     elseif ~isempty(regexp([trg_port_name_spltd{1} '_' trg_port_name_spltd{2} '_' ],'^DataServices_DCM_|^RoutineServices_DCM_','once'))||...
      |             ~isempty(regexp(trg_port_name_spltd{1},'^Dcm$','once'))
      |         TaskRate = '_dcmcb';
      |         
      |     %checking if this block is used under the function call trigger
      |     %starting with "Com" and then giving an error message
      |     %this is applicable only for APICALL
      |     elseif ~isempty(regexp(trg_port_name_spltd{1},'^Com$','once'))
      |         msg = sprintf(['\n','The Supplier call block "' Thisblk '" should not be present within APICALLs having function call trigger as "Com"']);
      |         errordlg(msg);
      |         return;
      |     end
      | end
      | 
      | DataName = ['Supplier_Call_Sepa_Main_Af_Po' TaskRate];%the variable name that should be given to DataStoreRead block 
      | set_param([Thisblk '/Data Store Read'],'DataStoreName',DataName);%Setting the DataStoreName of DataStoreRead block
      | 
      | %other settings done to this variable name
      | structVxx=Simulink.Signal;
      | structVxx.Dimensions=1;
      | structVxx.DimensionsMode='Fixed';
      | structVxx.DataType='single';
      | structVxx.Complexity='real';
      | structVxx.SamplingMode='Sample based';
      | structVxx.SampleTime=-1;
      | assignin('base',DataName,structVxx)
